simulink model "GFo_29bus"  (R2015b)
settings: Solver=ode1  StartTime=0.0  StopTime=4.5  FixedStep=Time_Step  RelTol=1e-3
PreLoadFcn:
  | Init_29bus;
InitFcn:
  | Init_29bus;
undefined symbols (not defined in the file): C_line, D1, D11, Delta, DX_DR, fb, fn, I_thresh_pu, Kp_Rvi_pu, Time_Step, VSC01_Cf, VSC01_Cf_pu, VSC01_Delta_P_Time_Step, VSC01_Delta_P_Value, VSC01_id0, VSC01_Lf, VSC01_Lf_pu, VSC01_Lt_pu, VSC01_mp1, VSC01_mp2, VSC01_mp3, VSC01_Pn, VSC01_R, VSC01_Rf, VSC01_Rf_pu, VSC01_Rt_pu, VSC01_Rv, VSC01_Sn, VSC01_T1, VSC01_T2, VSC01_Tr_PLL, VSC01_Udc_n, VSC01_Udcb, VSC01_Un1, VSC01_Un2, VSC01_W_LF, VSC01_wc1, VSC01_wc2, VSC01_wc3
libraries: powerlib x183, sps_avr x6, simulink x4, powerlib_meascontrol x2
(part 3 of 6)

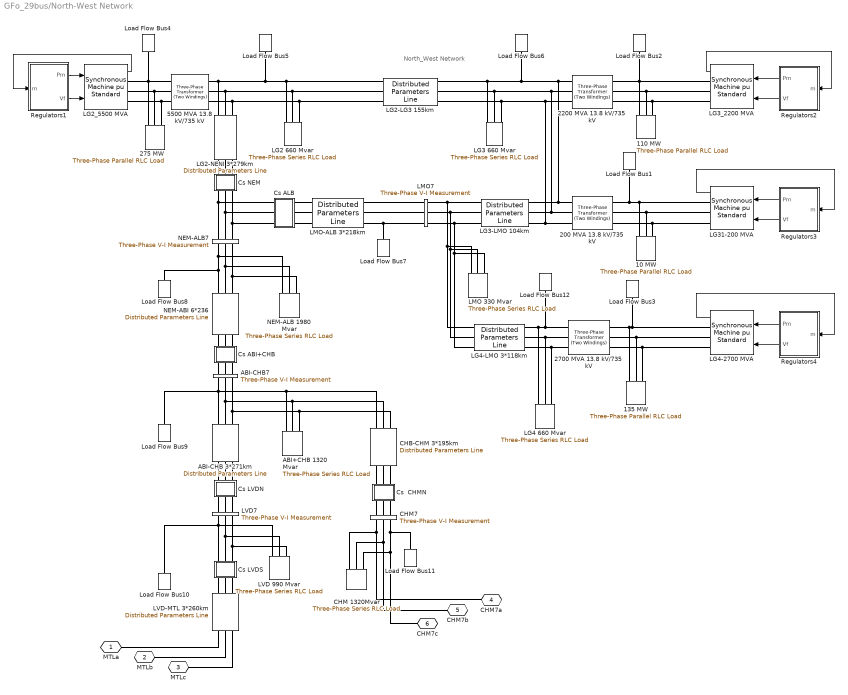
== system GFo_29bus/North-West Network ==
  note: North_West Network
  10 MW : powerlib/Elements/Three-Phase Parallel RLC Load  LConnTagsString=A|B|C  Configuration=Y (grounded)  NominalVoltage=(13800)*1  Vabc=[1e3 1e3 1e3]  Vabcp=[1e3 1e3 1e3]  NominalFrequency=60  UnbalancedPower=off  ActivePower=10000000  InductivePower=0  CapacitivePower=0  Pabc=[10e3 9e3 11e3]  QLabc=[100 90 110]  QCabc=[100 90 110]  Pabcp=[10e3 9e3 11e3]  QLabcp=[100 90 110]  QCabcp=[100 90 110]  Measurements=None  LoadType=constant PQ
  110 MW : powerlib/Elements/Three-Phase Parallel RLC Load  LConnTagsString=A|B|C  Configuration=Y (grounded)  NominalVoltage=(13800)*1  Vabc=[1e3 1e3 1e3]  Vabcp=[1e3 1e3 1e3]  NominalFrequency=60  UnbalancedPower=off  ActivePower=110000000  InductivePower=0  CapacitivePower=0  Pabc=[10e3 9e3 11e3]  QLabc=[100 90 110]  QCabc=[100 90 110]  Pabcp=[10e3 9e3 11e3]  QLabcp=[100 90 110]  QCabcp=[100 90 110]  Measurements=None  LoadType=constant PQ
  135 MW : powerlib/Elements/Three-Phase Parallel RLC Load  LConnTagsString=A|B|C  Configuration=Y (grounded)  NominalVoltage=(13800)*1  Vabc=[1e3 1e3 1e3]  Vabcp=[1e3 1e3 1e3]  NominalFrequency=60  UnbalancedPower=off  ActivePower=135000000  InductivePower=0  CapacitivePower=0  Pabc=[10e3 9e3 11e3]  QLabc=[100 90 110]  QCabc=[100 90 110]  Pabcp=[10e3 9e3 11e3]  QLabcp=[100 90 110]  QCabcp=[100 90 110]  Measurements=None  LoadType=constant PQ
  200 MVA 13.8 kV/735 kV : powerlib/Elements/Three-Phase Transformer (Two Windings)  Winding1Connection=Delta (D1)  Winding2Connection=Yg  CoreType=Three single-phase transformers  SetSaturation=off  Hysteresis=off  DataFile='basic_model'  SetInitialFlux=off  Measurements=None  UNITS=pu  NominalPower=[ 200e6 60 ]  Winding1="[ 13.8e3 0.002  0.0]"  Winding2=[ 735e3 0.002 0.12]  Rm=500  Lm=500  L0=0.5  Saturation="[ 0,0  ;  0.005,1.2  ;  1.0,1.4 ]"  InitialFluxes=[ 0.8 , -0.8 , 0.7 ]  MoreParameters=off  BreakLoop=off  DataType=off  TransfoNumber=0
  2200 MVA 13.8 kV/735 kV : powerlib/Elements/Three-Phase Transformer (Two Windings)  Winding1Connection=Delta (D1)  Winding2Connection=Yg  CoreType=Three single-phase transformers  SetSaturation=off  Hysteresis=off  DataFile='basic_model'  SetInitialFlux=off  Measurements=None  UNITS=pu  NominalPower=[ 2200e6 60 ]  Winding1="[ 13.8e3 0.002  0.0]"  Winding2=[ 735e3 0.002 0.12]  Rm=500  Lm=500  L0=0.5  Saturation="[ 0,0  ;  0.005,1.2  ;  1.0,1.4 ]"  InitialFluxes=[ 0.8 , -0.8 , 0.7 ]  MoreParameters=off  BreakLoop=off  DataType=off  TransfoNumber=0
  2700 MVA 13.8 kV/735 kV : powerlib/Elements/Three-Phase Transformer (Two Windings)  Winding1Connection=Delta (D1)  Winding2Connection=Yg  CoreType=Three single-phase transformers  SetSaturation=off  Hysteresis=off  DataFile='basic_model'  SetInitialFlux=off  Measurements=None  UNITS=pu  NominalPower=[ 2700e6 60 ]  Winding1="[ 13.8e3 0.002  0.0]"  Winding2=[ 735e3 0.002 0.12]  Rm=500  Lm=500  L0=0.5  Saturation="[ 0,0  ;  0.005,1.2  ;  1.0,1.4 ]"  InitialFluxes=[ 0.8 , -0.8 , 0.7 ]  MoreParameters=off  BreakLoop=off  DataType=off  TransfoNumber=0
  275 MW : powerlib/Elements/Three-Phase Parallel RLC Load  LConnTagsString=A|B|C  Configuration=Y (grounded)  NominalVoltage=(13800)*1  Vabc=[1e3 1e3 1e3]  Vabcp=[1e3 1e3 1e3]  NominalFrequency=60  UnbalancedPower=off  ActivePower=275000000  InductivePower=0  CapacitivePower=0  Pabc=[10e3 9e3 11e3]  QLabc=[100 90 110]  QCabc=[100 90 110]  Pabcp=[10e3 9e3 11e3]  QLabcp=[100 90 110]  QCabcp=[100 90 110]  Measurements=None  LoadType=constant PQ
  5500 MVA 13.8 kV/735 kV : powerlib/Elements/Three-Phase Transformer (Two Windings)  Winding1Connection=Delta (D1)  Winding2Connection=Yg  CoreType=Three single-phase transformers  SetSaturation=off  Hysteresis=off  DataFile='basic_model'  SetInitialFlux=off  Measurements=None  UNITS=pu  NominalPower=[ 5500e6 60 ]  Winding1="[ 13.8e3 0.002  0.0]"  Winding2=[ 735e3 0.002 0.12]  Rm=500  Lm=500  L0=0.5  Saturation="[ 0,0  ;  0.005,1.2  ;  1.0,1.4 ]"  InitialFluxes=[ 0.8 , -0.8 , 0.7 ]  MoreParameters=off  BreakLoop=off  DataType=off  TransfoNumber=0
  ABI+CHB 1320 Mvar : powerlib/Elements/Three-Phase Series RLC Load  LConnTagsString=A|B|C  Configuration=Y (grounded)  NominalVoltage=735e3  Vabc=[1e3 1e3 1e3]  Vabcp=[1e3 1e3 1e3]  NominalFrequency=60  UnbalancedPower=off  ActivePower=4400000  InductivePower=1320e6  CapacitivePower=0  Pabc=[10e3 9e3 11e3]  QLabc=[100 90 110]  QCabc=[100 90 110]  Pabcp=[10e3 9e3 11e3]  QLabcp=[100 90 110]  QCabcp=[100 90 110]  Measurements=None  LoadType=constant Z
  ABI-CHB 3*271km : powerlib/Elements/Distributed Parameters Line  Phases=3  Frequency=60  Resistance="[0.01273  0.3864]/3"  Inductance="[0.9337e-3  4.1264e-3]/3"  Capacitance=[12.74e-9 7.751e-9]*3  Length=271  x1=[-0.00156 -3.49602547978954e-08 0 0;-0.00152 -3.60388902575001e-08 0 0;-0.00148 -3.71093307842464e-08 0 0;-0.00144 -3.81713329691896e-08 0 0;-0.0014 -3.92246553221912e-08 0 0;-0.00136 -4.02690583268316e-08 0 0;-0.00132 -4.1304304494874e-08 0 0;-0.00128 -4.23301584202674e-08 0 0;-0.00124 -4.33463868326757e-08 0 0;-0.0012 -4.43527586505217e-08 0 0;-0.00116 -4.53490450335324e-08 0 0;-0.00112 -4.6335019434776e-08 0 0;-0.00108 -4.73104576521763e-08 0 0;-0.00104 -4.82751378794945e-08 0 0;-0.001 -4.9228840756766e-08 0 0;-0.00096 -5.01713494201809e-08 216587.676799688 -655260.200479363;-0.00092 -5.11024495513968e-08 226443.759556855 -651919.748758476;-0.00088 -5.20219294262736e-08 236248.350955866 -648431.056108637;-0.00084 -5.29295799630168e-08 245999.221517189 -644794.915828471;-0.0008 -5.38251947697217e-08 255694.153976947 -641012.15474492;-0.00076 -5.47085701913047e-08 265330.943791102 -637083.633025233;-0.00072 -5.55795053558128e-08 274907.399636756 -633010.243981371;-0.00068 -5.64378022201002e-08 284421.343910432 -628792.913866876;-0.00064 -5.72832656148616e-08 293870.613223249 -624432.601666247;-0.0006 -5.81157032890121e-08 303253.058892851 -619930.298876876;-0.00056 -5.89349259534031e-08 312566.547432004 -615287.029283592;-0.00052 -5.97407473238655e-08 321808.96103373 -610503.848725858;-0.00048 -6.05329841635687e-08 330978.198052879 -605581.844857685;-0.00044 -6.13114563246873e-08 340072.173484025 -600522.136900307;-0.0004 -6.20759867893652e-08 349088.819435579 -595325.87538768;-0.00036 -6.28264017099676e-08 358026.085600006 -589994.241904861;-0.00032 -6.35625304486131e-08 366881.939720054 -584528.448819327;-0.00028 -6.42842056159744e-08 375654.368050865 -578929.73900529;-0.00024 -6.49912631093421e-08 384341.375817886 -573199.38556108;-0.0002 -6.56835421499394e-08 392940.987670464 -567338.691519655;-0.00016 -6.63608853194826e-08 401451.248131026 -561348.989552299;-0.00012 -6.70231385959761e-08 409870.22203973 -555231.641665587;-8e-05 -6.76701513887358e-08 418195.994994513 -548988.038891673;-4e-05 -6.83017765726322e-08 426426.673786403 -542619.600971986]  x2=[-0.00156 -7.66036881931219e-08 0 0;-0.00152 -7.88179038071448e-08 0 0;-0.00148 -8.10141969095385e-08 0 0;-0.00144 -8.31920680821918e-08 0 0;-0.0014 -8.53510220959809e-08 0 0;-0.00136 -8.74905680233813e-08 0 0;-0.00132 -8.96102193500997e-08 0 0;-0.00128 -9.17094940857036e-08 0 0;-0.00124 -9.37879148732213e-08 0 0;-0.0012 -9.58450090976894e-08 0 0;-0.00116 -9.78803089936208e-08 0 0;-0.00112 -9.98933517513709e-08 0 0;-0.00108 -1.01883679622376e-07 0 0;-0.00104 -1.03850840023243e-07 0 0;-0.001 -1.0579438563866e-07 0 0;-0.00096 -1.07713874523115e-07 -50356.5060781829 -677474.330127236;-0.00092 -1.09608870201388e-07 -40135.0993416283 -678156.632405211;-0.00088 -1.11478941767803e-07 -29904.5662295937 -678684.727713151;-0.00084 -1.13323663984215e-07 -19667.2330770844 -679058.495966737;-0.0008 -1.15142617376698e-07 -9425.42776537653 -679277.852174291;-0.00076 -1.16935388330937e-07 818.520807323877 -679342.746456104;-0.00072 -1.18701569186277e-07 11062.2832554513 -679253.164055774;-0.00068 -1.20440758328423e-07 21303.5302357635 -679009.125343568;-0.00064 -1.22152560280763e-07 31539.9329770139 -678610.685811785;-0.0006 -1.23836585794293e-07 41769.1638094941 -678057.936062137;-0.00056 -1.25492451936135e-07 51988.8966943259 -677351.001785151;-0.00052 -1.27119782176607e-07 62196.8077523827 -676490.043731585;-0.00048 -1.28718206474847e-07 72390.5757927189 -675475.257675877;-0.00044 -1.30287361362953e-07 82567.8828403897 -674306.874371624;-0.0004 -1.31826890028635e-07 92726.4146635376 -672985.159499113;-0.00036 -1.33336442396351e-07 102863.86129963 -671510.413604909;-0.00032 -1.34815675206911e-07 112977.917580722 -669882.972033511;-0.00028 -1.3626425209553e-07 123066.283657637 -668103.204851096;-0.00024 -1.37681843668315e-07 133126.665522926 -666171.516761376;-0.0002 -1.39068127577168e-07 143156.775532512 -664088.347013562;-0.00016 -1.40422788593082e-07 153154.332925872 -661854.169302491;-0.00012 -1.41745518677825e-07 163117.064344672 -659469.491660909;-8e-05 -1.43036017053981e-07 173042.704349701 -656934.856343945;-4e-05 -1.4429399027335e-07 182928.995936018 -654250.839705814]  x3=[-0.00156 3.89449950371453e-10 0 0;-0.00152 3.78955368381599e-10 0 0;-0.00148 3.68374615208948e-10 0 0;-0.00144 3.57710096825525e-10 0 0;-0.0014 3.46964238250845e-10 0 0;-0.00136 3.36139483000479e-10 0 0;-0.00132 3.25238292530421e-10 0 0;-0.00128 3.14263145677378e-10 0 0;-0.00124 3.03216538095098e-10 0 0;-0.0012 2.92100981686883e-10 0 0;-0.00116 2.80919004034404e-10 0 0;-0.00112 2.6967314782295e-10 0 0;-0.00108 2.58365970263243e-10 0 0;-0.00104 2.47000042509952e-10 0 0;-0.001 2.35577949077031e-10 0 0;-0.00096 2.24102287250028e-10 85.100387182329 865.220294474964;-0.00092 2.1257566649548e-10 72.0441612628443 866.405402860482;-0.00088 2.01000707867546e-10 58.9715531223708 867.393498128952;-0.00084 1.89380043411998e-10 45.8855353592663 868.18435559603;-0.0008 1.77716315567723e-10 32.7890836211211 868.777795427549;-0.00076 1.66012176565848e-10 19.6851759281215 869.173682680408;-0.00072 1.5427028782665e-10 6.57679199587353 869.37192733326;-0.00068 1.4249331935437e-10 -6.53308744215846 869.37248430698;-0.00064 1.3068394913008e-10 -19.6414813124451 869.175353474919;-0.0006 1.18844862502727e-10 -32.7454088792621 868.780579662926;-0.00056 1.06978751578516e-10 -45.8418904224844 868.188252639162;-0.00052 9.50883146087413e-11 -58.9279479151482 867.398507093685;-0.00048 8.31762553762313e-11 -72.0006057006291 866.411522607821;-0.00044 7.12452825805302e-11 -85.0568911692805 865.227523613331;-0.0004 5.92981092219635e-11 -98.0938354343793 863.846779341375;-0.00036 4.73374519847248e-11 -111.108474007226 862.269603761295;-0.00032 3.53660306191255e-11 -124.097847471241 860.496355509215;-0.00028 2.33865673231472e-11 -137.059002154916 858.527437806497;-0.00024 1.14017861234367e-11 -149.988990803448 856.363298368048;-0.0002 -5.85587744113456e-13 -162.884873248921 854.004429300512;-0.00016 -1.25728284540605e-11 -175.743717078876 851.451366990373;-0.00012 -2.45572102112405e-11 -188.562598303117 848.704691981985;-8e-05 -3.65360078705908e-11 -201.338602018598 845.765028845558;-4e-05 -4.85064975568245e-11 -214.06882307225 842.633046035138]  x4=[-0.00156 -5.54020599902801e-10 0 0;-0.00152 -5.57562391334411e-10 0 0;-0.00148 -5.60977397886446e-10 0 0;-0.00144 -5.64264843015864e-10 0 0;-0.0014 -5.67423979185994e-10 0 0;-0.00136 -5.70454088036512e-10 0 0;-0.00132 -5.73354480546798e-10 0 0;-0.00128 -5.76124497192605e-10 0 0;-0.00124 -5.78763508096037e-10 0 0;-0.0012 -5.81270913168772e-10 0 0;-0.00116 -5.83646142248519e-10 0 0;-0.00112 -5.85888655228669e-10 0 0;-0.00108 -5.87997942181109e-10 0 0;-0.00104 -5.89973523472174e-10 0 0;-0.001 -5.91814949871717e-10 0 0;-0.00096 -5.93521802655255e-10 -873.234445044949 -15818.0204896519;-0.00092 -5.95093693699182e-10 -634.614399883324 -15829.3897607238;-0.00088 -5.96530265569031e-10 -395.850048879845 -15837.1595650709;-0.00084 -5.97831191600748e-10 -156.995684988917 -15841.3281359068;-0.0008 -5.98996175974972e-10 81.8943783669032 -15841.8945253344;-0.00076 -6.00024953784302e-10 320.765819647312 -15838.8586045616;-0.00072 -6.00917291093536e-10 559.564321546497 -15832.2210639306;-0.00068 -6.01672984992866e-10 798.235583344441 -15821.983412761;-0.00064 -6.02291863644015e-10 1036.72533325442 -15808.1479790062;-0.0006 -6.02773786319315e-10 1274.97934076396 -15790.7179087247;-0.00056 -6.03118643433706e-10 1512.94342896636 -15769.6971653641;-0.00052 -6.03326356569654e-10 1750.56348688009 -15745.0905288602;-0.00048 -6.03396878494983e-10 1987.78548175311 -15716.9035945499;-0.00044 -6.03330193173615e-10 2224.55547134952 -15685.142771899;-0.0004 -6.03126315769217e-10 2460.81961621549 -15649.8152830446;-0.00036 -6.02785292641754e-10 2696.52419192193 -15610.9291611532;-0.00032 -6.02307201336942e-10 2931.61560128097 -15568.4932485934;-0.00028 -6.01692150568623e-10 3166.04038653345 -15522.5171949259;-0.00024 -6.00940280194036e-10 3399.74524150481 -15473.0114547087;-0.0002 -6.00051761182022e-10 3632.6770237264 -15419.9872851203;-0.00016 -5.99026795574141e-10 3864.78276651966 -15363.4567433996;-0.00012 -5.97865616438733e-10 4096.00969104029 -15303.4326841042;-8e-05 -5.96568487817921e-10 4326.30521827966 -15239.9287561877;-4e-05 -5.95135704667566e-10 4555.61698102086 -15172.9593998955]  x5=0.00153261764655846  V1=ones(3,3)  V2=ones(3,3)  I1=ones(3,3)  I2=ones(3,3)  nHarmo=1  Measurements=None
      settings: AttributesFormatString=\n
  ABI-CHB7 : powerlib/Measurements/Three-Phase V-I Measurement  VoltageMeasurement=no  SetLabelV=on  LabelV=Vabc_ABI7  Vpu=on  VpuLL=off  CurrentMeasurement=no  SetLabelI=off  LabelI=A1  Ipu=off  Pbase=100e6  Vbase=500e3  OutputType=Magnitude  PhasorSimulation=off  PSBequivalent=0
  CHB-CHM 3*195km : powerlib/Elements/Distributed Parameters Line  Phases=3  Frequency=60  Resistance="[0.01273  0.3864]/3"  Inductance="[0.9337e-3  4.1264e-3]/3"  Capacitance=[12.74e-9 7.751e-9]*3  Length=195  x1=[-0.00112 -4.6335019434776e-08 0 0;-0.00108 -4.73104576521763e-08 0 0;-0.00104 -4.82751378794945e-08 0 0;-0.001 -4.9228840756766e-08 0 0;-0.00096 -5.01713494201809e-08 0 0;-0.00092 -5.11024495513968e-08 0 0;-0.00088 -5.20219294262736e-08 0 0;-0.00084 -5.29295799630168e-08 0 0;-0.0008 -5.38251947697217e-08 0 0;-0.00076 -5.47085701913047e-08 0 0;-0.00072 -5.55795053558128e-08 0 0;-0.00068 -5.64378022201002e-08 284421.343910432 -628792.913866876;-0.00064 -5.72832656148616e-08 293870.613223249 -624432.601666247;-0.0006 -5.81157032890121e-08 303253.058892851 -619930.298876876;-0.00056 -5.89349259534031e-08 312566.547432004 -615287.029283592;-0.00052 -5.97407473238655e-08 321808.96103373 -610503.848725858;-0.00048 -6.05329841635687e-08 330978.198052879 -605581.844857685;-0.00044 -6.13114563246873e-08 340072.173484025 -600522.136900307;-0.0004 -6.20759867893652e-08 349088.819435579 -595325.87538768;-0.00036 -6.28264017099676e-08 358026.085600006 -589994.241904861;-0.00032 -6.35625304486131e-08 366881.939720054 -584528.448819327;-0.00028 -6.42842056159744e-08 375654.368050865 -578929.73900529;-0.00024 -6.49912631093421e-08 384341.375817886 -573199.38556108;-0.0002 -6.56835421499394e-08 392940.987670464 -567338.691519655;-0.00016 -6.63608853194826e-08 401451.248131026 -561348.989552299;-0.00012 -6.70231385959761e-08 409870.22203973 -555231.641665587;-8e-05 -6.76701513887358e-08 418195.994994513 -548988.038891673;-4e-05 -6.83017765726322e-08 426426.673786403 -542619.600971986]  x2=[-0.00112 -3.4035079791735e-08 0 0;-0.00108 -3.46803398916117e-08 0 0;-0.00104 -3.53177139812674e-08 0 0;-0.001 -3.59470571273309e-08 0 0;-0.00096 -3.65682262225978e-08 0 0;-0.00092 -3.71810800185726e-08 0 0;-0.00088 -3.77854791575872e-08 0 0;-0.00084 -3.83812862044894e-08 0 0;-0.0008 -3.89683656778949e-08 0 0;-0.00076 -3.95465840809941e-08 0 0;-0.00072 -4.01158099319085e-08 0 0;-0.00068 -4.06759137935883e-08 200688.40467491 -641039.156089466;-0.00064 -4.12267683032457e-08 210331.860760861 -637940.078467723;-0.0006 -4.17682482013154e-08 219927.4891955 -634695.938773497;-0.00056 -4.23002303599382e-08 229473.108015669 -631307.474696179;-0.00052 -4.28225938109587e-08 238966.546629967 -627775.456743278;-0.00048 -4.3335219773433e-08 248405.646312322 -624100.68806522;-0.00044 -4.38379916806378e-08 257788.260692864 -620284.00427271;-0.0004 -4.43307952065771e-08 267112.256245996 -616326.27324673;-0.00036 -4.4813518291979e-08 276375.512775535 -612228.394941185;-0.00032 -4.52860511697766e-08 285575.92389683 -607991.301178263;-0.00028 -4.57482863900685e-08 294711.397515733 -603615.955436548;-0.00024 -4.62001188445517e-08 303779.856304324 -599103.352631928;-0.0002 -4.66414457904225e-08 312779.238173277 -594454.518891367;-0.00016 -4.70721668737393e-08 321707.496740762 -589670.511319567;-0.00012 -4.7492184152242e-08 330562.601797777 -584752.417758595;-8e-05 -4.79014021176237e-08 339342.539769792 -579701.356540515;-4e-05 -4.82997277172479e-08 348045.31417463 -574518.47623309]  x3=[-0.00112 -2.96726562445571e-10 0 0;-0.00108 -2.98557921265796e-10 0 0;-0.00104 -3.00321390589379e-10 0 0;-0.001 -3.02016569418604e-10 0 0;-0.00096 -3.03643072284422e-10 0 0;-0.00092 -3.0520052933411e-10 0 0;-0.00088 -3.06688586415364e-10 0 0;-0.00084 -3.08106905156837e-10 0 0;-0.0008 -3.09455163045078e-10 0 0;-0.00076 -3.1073305349787e-10 0 0;-0.00072 -3.11940285933945e-10 0 0;-0.00068 -3.13076585839056e-10 1577.00475277505 -3661.5344585744;-0.00064 -3.14141694828406e-10 1632.03842707261 -3637.33809003913;-0.0006 -3.15135370705393e-10 1686.70098990594 -3612.31462218926;-0.00056 -3.16057387516695e-10 1740.98001147967 -3586.46974514558;-0.00052 -3.16907535603638e-10 1794.86314921235 -3559.80933581025;-0.00048 -3.17685621649878e-10 1848.33815054315 -3532.33945653044;-0.00044 -3.1839146872536e-10 1901.3928557179 -3504.06635371982;-0.0004 -3.19024916326544e-10 1954.01520055417 -3474.99645643815;-0.00036 -3.1958582041291e-10 2006.19321918455 -3445.13637492937;-0.00032 -3.20074053439705e-10 2057.91504677755 -3414.49289911852;-0.00028 -3.20489504386948e-10 2109.16892223563 -3383.07299706775;-0.00024 -3.20832078784677e-10 2159.94319086948 -3350.88381339182;-0.0002 -3.21101698734429e-10 2210.22630704829 -3317.93266763352;-0.00016 -3.21298302926952e-10 2260.00683682506 -3284.22705259923;-0.00012 -3.21421846656148e-10 2309.2734605366 -3249.77463265515;-8e-05 -3.21472301829238e-10 2358.01497537754 -3214.58324198447;-4e-05 -3.21449656973151e-10 2406.22029794773 -3178.66088280594]  x4=[-0.00112 7.78404396619644e-11 0 0;-0.00108 7.25066391557828e-11 0 0;-0.00104 6.71563512651278e-11 0 0;-0.001 6.17907925993268e-11 0 0;-0.00096 5.64111832401498e-11 0 0;-0.00092 5.10187464643733e-11 0 0;-0.00088 4.56147084656178e-11 0 0;-0.00084 4.02002980755216e-11 0 0;-0.0008 3.47767464843158e-11 0 0;-0.00076 2.93452869608612e-11 0 0;-0.00072 2.39071545722147e-11 0 0;-0.00068 1.84635859027851e-11 1976.43464506423 -10995.3468033902;-0.00064 1.30158187731443e-11 2142.0090164811 -10964.2940798932;-0.0006 7.56509195855814e-12 2307.09631351953 -10930.7481704745;-0.00056 2.11264490729919e-12 2471.65899675181 -10894.7167031845;-0.00052 -3.34028254119301e-12 2635.65964604292 -10856.2078712683;-0.00048 -8.79245043824072e-12 2799.06096905947 -10815.2304313021;-0.00044 -1.42426190078816e-11 2961.82580974973 -10771.7937012024;-0.0004 -1.96895489287832e-11 3123.91715679255 -10725.9075581071;-0.00036 -2.51320016160539e-11 3285.29815201344 -10677.5824361293;-0.00032 -3.05687395028862e-11 3445.93209876576 -10626.8293239851;-0.00028 -3.59985263219692e-11 3605.78247027527 -10573.6597624945;-0.00024 -4.14201273866046e-11 3764.81291794598 -10518.0858419572;-0.0002 -4.68323098714643e-11 3922.98727962552 -10460.1201994036;-0.00016 -5.22338430929238e-11 4080.26958782808 -10399.7760157209;-0.00012 -5.76234987889094e-11 4236.6240779131 -10337.0670126561;-8e-05 -6.30000513981944e-11 4392.0151962179 -10272.0074496957;-4e-05 -6.83622783390807e-11 4546.40760814221 -10204.6121208232]  x5=0.0011028060556417  V1=ones(3,3)  V2=ones(3,3)  I1=ones(3,3)  I2=ones(3,3)  nHarmo=1  Measurements=None
      settings: AttributesFormatString=\n
  CHM 1320Mvar : powerlib/Elements/Three-Phase Series RLC Load  LConnTagsString=A|B|C  Configuration=Y (grounded)  NominalVoltage=735e3  Vabc=[1e3 1e3 1e3]  Vabcp=[1e3 1e3 1e3]  NominalFrequency=60  UnbalancedPower=off  ActivePower=4400000  InductivePower=1320e6  CapacitivePower=0  Pabc=[10e3 9e3 11e3]  QLabc=[100 90 110]  QCabc=[100 90 110]  Pabcp=[10e3 9e3 11e3]  QLabcp=[100 90 110]  QCabcp=[100 90 110]  Measurements=None  LoadType=constant Z
  CHM7 : powerlib/Measurements/Three-Phase V-I Measurement  VoltageMeasurement=no  SetLabelV=on  LabelV=Vabc_CHM7  Vpu=on  VpuLL=off  CurrentMeasurement=no  SetLabelI=off  LabelI=A1  Ipu=off  Pbase=100e6  Vbase=735e3  OutputType=Magnitude  PhasorSimulation=off  PSBequivalent=0
  "Cs  CHMN " : Subsystem  mask{Xc=25/3}
      mask prompts: Xc "Condensator Reactance at  60Hz  (ohm):"
      mask help: Series Compensation
      mask init:
      | Cs=1/Xc/(2*pi*60);
      mask Display: disp('Cs')
  "Cs ABI+CHB " : Subsystem  mask{Xc=25/6}
      mask prompts: Xc "Condensator Reactance at  60Hz  (ohm):"
      mask help: Series Compensation
      mask init:
      | Cs=1/Xc/(2*pi*60);
      mask Display: disp('Cs')
  Cs ALB : Subsystem  mask{Xc=16/3}
      mask prompts: Xc "Reactance @ 60Hz du condensateur (ohm):"
      mask init:
      | Cs=1/Xc/(2*pi*60);
      mask Display: disp('Cs')
  "Cs LVDN " : Subsystem  mask{Xc=34/3}
      mask prompts: Xc "Condensator Reactance at  60Hz  (ohm):"
      mask help: Series Compensation
      mask init:
      | Cs=1/Xc/(2*pi*60);
      mask Display: disp('Cs')
  "Cs LVDS " : Subsystem  mask{Xc=34/3}
      mask prompts: Xc "Condensator Reactance at  60Hz  (ohm):"
      mask help: Series Compensation
      mask init:
      | Cs=1/Xc/(2*pi*60);
      mask Display: disp('Cs')
  "Cs NEM " : Subsystem  mask{Xc=16/3}
      mask prompts: Xc "Condensator Reactance at  60Hz  (ohm):"
      mask help: Series Compensation
      mask init:
      | Cs=1/Xc/(2*pi*60);
      mask Display: disp('Cs')
  LG2 660 Mvar : powerlib/Elements/Three-Phase Series RLC Load  LConnTagsString=A|B|C  Configuration=Y (grounded)  NominalVoltage=735e3  Vabc=[1e3 1e3 1e3]  Vabcp=[1e3 1e3 1e3]  NominalFrequency=60  UnbalancedPower=off  ActivePower=2200000  InductivePower=660e6  CapacitivePower=0  Pabc=[10e3 9e3 11e3]  QLabc=[100 90 110]  QCabc=[100 90 110]  Pabcp=[10e3 9e3 11e3]  QLabcp=[100 90 110]  QCabcp=[100 90 110]  Measurements=None  LoadType=constant Z
  LG2-LG3 155km : powerlib/Elements/Distributed Parameters Line  Phases=3  Frequency=60  Resistance="[0.01273  0.3864]"  Inductance="[0.9337e-3  4.1264e-3]"  Capacitance=[12.74e-9 7.751e-9]  Length=155  x1=[-0.00088 -4.23262671580693e-09 492217.122941526 -498797.252764154;-0.00084 -4.28940865142763e-09 499682.540946216 -491318.32934528;-0.0008 -4.34521521251128e-09 507034.335450174 -483727.684375262;-0.00076 -4.40003370912715e-09 514270.834718728 -476027.043901306;-0.00072 -4.45385167602183e-09 521390.39323435 -468218.15898265;-0.00068 -4.50665687545377e-09 528391.39207083 -460302.805292382;-0.00064 -4.55843729997599e-09 535272.239261406 -452282.782713673;-0.0006 -4.60918117516648e-09 542031.370160766 -444159.914930496;-0.00056 -4.65887696230562e-09 548667.24780083 -435936.049012936;-0.00052 -4.70751336099998e-09 555178.363240249 -427613.054997182;-0.00048 -4.75507931175191e-09 561563.235907522 -419192.8254603;-0.00044 -4.80156399847441e-09 567820.413937664 -410677.275089874;-0.0004 -4.84695685095058e-09 573948.474502352 -402068.340248621;-0.00036 -4.89124754723722e-09 579946.024133459 -393367.978534086;-0.00032 -4.93442601601193e-09 585811.699039919 -384578.168333494;-0.00028 -4.97648243886329e-09 591544.165417842 -375700.908373883;-0.00024 -5.01740725252341e-09 597142.119753809 -366738.217267614;-0.0002 -5.05719115104257e-09 602604.289121279 -357692.133053355;-0.00016 -5.09582508790535e-09 607929.43147004 -348564.712732645;-0.00012 -5.13330027808767e-09 613116.335908645 -339358.031802154;-8e-05 -5.16960820005444e-09 618163.822979755 -330074.183781729;-4e-05 -5.20474059769733e-09 623070.744928336 -320715.279738352]  x2=[-0.00088 -6.68954234344848e-09 498836.623614221 -488147.5029039;-0.00084 -6.77458910534282e-09 506140.702918543 -480569.9805379;-0.0008 -6.85809538409617e-09 513329.690191792 -472883.180702585;-0.00076 -6.94004219110087e-09 520401.950720259 -465088.851309949;-0.00072 -7.0204108923597e-09 527355.876332888 -457188.764723281;-0.00068 -7.09918321272305e-09 534189.885766961 -449184.717354143;-0.00064 -7.17634124004457e-09 540902.425027669 -441078.529253882;-0.0006 -7.25186742925423e-09 547491.967741469 -432872.043699768;-0.00056 -7.32574460634793e-09 553957.015503175 -424567.126775847;-0.00052 -7.39795597229267e-09 560296.098216677 -416165.666948607;-0.00048 -7.46848510684657e-09 566507.774429232 -407669.574637564;-0.00044 -7.53731597229265e-09 572590.631659237 -399080.78178084;-0.0004 -7.60443291708567e-09 578543.286717413 -390401.241395866;-0.00036 -7.66982067941118e-09 584364.386021336 -381632.927135275;-0.00032 -7.73346439065591e-09 590052.60590322 -372777.832838115;-0.00028 -7.79534957878876e-09 595606.65291092 -363837.972076468;-0.00024 -7.85546217165163e-09 601025.26410204 -354815.377697575;-0.0002 -7.91378850015928e-09 606307.207331125 -345712.101361591;-0.00016 -7.9703153014076e-09 611451.281529833 -336530.213075052;-0.00012 -8.02502972168946e-09 616456.316980053 -327271.800720173;-8e-05 -8.0779193194175e-09 621321.175579884 -317938.969580082;-4e-05 -8.12897206795333e-09 626044.751102434 -308533.841860097]  x3=[-0.00088 1.32376578464899e-12 1822.53525045153 -2130.11317243652;-0.00084 1.08156186492231e-12 1854.44819935546 -2102.38868894714;-0.0008 8.39112007354538e-13 1885.93946273093 -2074.18614040013;-0.00076 5.96471342952486e-13 1917.00187973622 -2045.5119398118;-0.00072 3.53695046110797e-13 1947.62838704559 -2016.37260744811;-0.00068 1.10838322065759e-13 1977.81202045537 -1986.77476934194;-0.00064 -1.3204360565789e-13 2007.54591646762 -1956.72515578643;-0.0006 -3.74895507804306e-13 2036.82331385081 -1926.23059980458;-0.00056 -6.1766216194521e-13 2065.63755517724 -1895.29803559544;-0.00052 -8.60288365036977e-13 2093.98208833693 -1863.93449695736;-0.00048 -1.10271894597335e-12 2121.85046802746 -1832.14711568856;-0.00044 -1.34489877813085e-12 2149.23635721962 -1799.94311996541;-0.0004 -1.58677279190411e-12 2176.13352859837 -1767.32983269884;-0.00036 -1.82828598722824e-12 2202.5358659789 -1734.3146698691;-0.00032 -2.06938344608534e-12 2228.43736569736 -1700.90513883954;-0.00028 -2.31001034499241e-12 2253.83213797609 -1667.10883664938;-0.00024 -2.5501119674677e-12 2278.71440826287 -1632.93344828631;-0.0002 -2.78963371647283e-12 2303.078518544 -1598.38674493891;-0.00016 -3.0285211268276e-12 2326.91892863091 -1563.47658222961;-0.00012 -3.26671987759499e-12 2350.23021741996 -1528.21089842836;-8e-05 -3.5041758044332e-12 2373.00708412508 -1492.59771264754;-4e-05 -3.74083491191221e-12 2395.24434948321 -1456.64512301848]  x4=[-0.00088 -1.27329221211409e-11 1450.99532516357 -1864.39271134758;-0.00084 -1.27177947276358e-11 1478.94347975619 -1842.30101377444;-0.0008 -1.26997754172833e-11 1506.55533535538 -1819.79039283809;-0.00076 -1.26788682875191e-11 1533.82461326329 -1796.86596725961;-0.00072 -1.26550780924442e-11 1560.74511268128 -1773.5329498557;-0.00068 -1.26284102417439e-11 1587.31071211994 -1749.79664635328;-0.00064 -1.25988707994573e-11 1613.51537079105 -1725.66245418308;-0.0006 -1.2566466482599e-11 1639.35312998121 -1701.13586125228;-0.00056 -1.25312046596311e-11 1664.81811440679 -1676.22244469661;-0.00052 -1.24930933487881e-11 1689.90453354993 -1650.92786961213;-0.00048 -1.24521412162535e-11 1714.60668297526 -1625.25788776711;-0.00044 -1.2408357574189e-11 1738.91894562702 -1599.21833629403;-0.0004 -1.23617523786172e-11 1762.83579310634 -1572.81513636235;-0.00036 -1.23123362271578e-11 1786.35178692836 -1546.05429183204;-0.00032 -1.22601203566173e-11 1809.46157975887 -1518.94188788837;-0.00028 -1.22051166404346e-11 1832.15991663028 -1491.48408965819;-0.00024 -1.21473375859802e-11 1854.44163613651 -1463.68714080804;-0.0002 -1.2086796331713e-11 1876.30167160672 -1435.55736212437;-0.00016 -1.2023506644192e-11 1897.73505225734 -1407.10115007627;-0.00012 -1.19574829149465e-11 1918.73690432244 -1378.32497536096;-8e-05 -1.1888740157203e-11 1939.30245216199 -1349.23538143243;-4e-05 -1.18172940024719e-11 1959.42701934774 -1319.83898301347]  x5=0.000876589428843401  V1=ones(3,3)  V2=ones(3,3)  I1=ones(3,3)  I2=ones(3,3)  nHarmo=1  Measurements=None
      settings: AttributesFormatString=\n
  LG2-NENI 3*279km : powerlib/Elements/Distributed Parameters Line  Phases=3  Frequency=60  Resistance="[0.01273  0.3864]/3"  Inductance="[0.9337e-3  4.1264e-3]/3"  Capacitance=[12.74e-9 7.751e-9]*3  Length=279  x1=[-0.0016 -3.05949440922947e-09 0 0;-0.00156 -3.13142523515607e-09 0 0;-0.00152 -3.20264400198844e-09 0 0;-0.00148 -3.2731345151932e-09 0 0;-0.00144 -3.3428807458355e-09 0 0;-0.0014 -3.41186683422398e-09 0 0;-0.00136 -3.48007709351705e-09 0 0;-0.00132 -3.54749601328995e-09 0 0;-0.00128 -3.61410826306174e-09 0 0;-0.00124 -3.67989869578125e-09 0 0;-0.0012 -3.74485235127143e-09 0 0;-0.00116 -3.80895445963116e-09 0 0;-0.00112 -3.8721904445938e-09 0 0;-0.00108 -3.93454592684169e-09 0 0;-0.00104 -3.99600672727588e-09 0 0;-0.001 -4.0565588702404e-09 469156.230502968 -520546.816624002;-0.00096 -4.11618858670009e-09 476952.23216764 -513413.158168939;-0.00092 -4.17488231737167e-09 484639.779007779 -506162.753989194;-0.00088 -4.23262671580693e-09 492217.122941526 -498797.252764154;-0.00084 -4.28940865142763e-09 499682.540946216 -491318.32934528;-0.0008 -4.34521521251128e-09 507034.335450174 -483727.684375262;-0.00076 -4.40003370912715e-09 514270.834718728 -476027.043901306;-0.00072 -4.45385167602183e-09 521390.39323435 -468218.15898265;-0.00068 -4.50665687545377e-09 528391.39207083 -460302.805292382;-0.00064 -4.55843729997599e-09 535272.239261406 -452282.782713673;-0.0006 -4.60918117516648e-09 542031.370160766 -444159.914930496;-0.00056 -4.65887696230562e-09 548667.24780083 -435936.049012936;-0.00052 -4.70751336099998e-09 555178.363240249 -427613.054997182;-0.00048 -4.75507931175191e-09 561563.235907522 -419192.8254603;-0.00044 -4.80156399847441e-09 567820.413937664 -410677.275089874;-0.0004 -4.84695685095058e-09 573948.474502352 -402068.340248621;-0.00036 -4.89124754723722e-09 579946.024133459 -393367.978534086;-0.00032 -4.93442601601193e-09 585811.699039919 -384578.168333494;-0.00028 -4.97648243886329e-09 591544.165417842 -375700.908373883;-0.00024 -5.01740725252341e-09 597142.119753809 -366738.217267614;-0.0002 -5.05719115104257e-09 602604.289121279 -357692.133053355;-0.00016 -5.09582508790535e-09 607929.43147004 -348564.712732645;-0.00012 -5.13330027808767e-09 613116.335908645 -339358.031802154;-8e-05 -5.16960820005444e-09 618163.822979755 -330074.183781729;-4e-05 -5.20474059769733e-09 623070.744928336 -320715.279738352]  x2=[-0.0016 -2.24433015141576e-08 0 0;-0.00156 -2.31214987165789e-08 0 0;-0.00152 -2.37944382895833e-08 0 0;-0.00148 -2.44619672125152e-08 0 0;-0.00144 -2.5123933695054e-08 0 0;-0.0014 -2.57801872117301e-08 0 0;-0.00136 -2.64305785361532e-08 0 0;-0.00132 -2.70749597749447e-08 0 0;-0.00128 -2.77131844013679e-08 0 0;-0.00124 -2.83451072886465e-08 0 0;-0.0012 -2.89705847429655e-08 0 0;-0.00116 -2.95894745361457e-08 0 0;-0.00112 -3.02016359379851e-08 0 0;-0.00108 -3.080692974826e-08 0 0;-0.00104 -3.14052183283778e-08 0 0;-0.001 -3.19963656326748e-08 282230.706828565 -628834.165902495;-0.00096 -3.25802372393518e-08 291680.843809443 -624506.879482045;-0.00092 -3.31567003810406e-08 301064.655081788 -620037.585582718;-0.00088 -3.37256239749939e-08 310380.006847838 -615427.300483406;-0.00084 -3.42868786528928e-08 319624.780876934 -610677.072523183;-0.0008 -3.48403367902634e-08 328796.874987185 -605787.981862923;-0.00076 -3.53858725354982e-08 337894.203523488 -600761.140239681;-0.00072 -3.59233618384731e-08 346914.697831784 -595597.690713891;-0.00068 -3.64526824787559e-08 355856.306729459 -590298.807409449;-0.00064 -3.69737140933976e-08 364716.996971758 -584865.695246722;-0.0006 -3.74863382043021e-08 373494.753714131 -579299.589668563;-0.00056 -3.79904382451674e-08 382187.580970391 -573601.756359381;-0.00052 -3.84858995879914e-08 390793.502066583 -567773.490957332;-0.00048 -3.89726095691373e-08 399310.560090465 -561816.118759711;-0.00044 -3.94504575149526e-08 407736.81833649 -555730.994421579;-0.0004 -3.99193347669353e-08 416070.360746198 -549519.501647736;-0.00036 -4.03791347064417e-08 424309.292343911 -543183.052878072;-0.00032 -4.08297527789307e-08 432451.739667631 -536723.088966395;-0.00028 -4.12710865177385e-08 440495.851195057 -530141.07885279;-0.00024 -4.17030355673789e-08 448439.797764595 -523438.519229596;-0.0002 -4.21255017063629e-08 456281.772991301 -516616.93420107;-0.00016 -4.25383888695337e-08 464019.993677636 -509677.874936822;-0.00012 -4.29416031699111e-08 471652.700218946 -502622.919319088;-8e-05 -4.33350529200402e-08 479178.157003586 -495453.671583936;-4e-05 -4.37186486528409e-08 486594.65280758 -488171.761956477]  x3=[-0.0016 2.26069456197243e-10 0 0;-0.00156 2.22950163037741e-10 0 0;-0.00152 2.19780172933805e-10 0 0;-0.00148 2.16560206713847e-10 0 0;-0.00144 2.13290996570417e-10 0 0;-0.0014 2.09973285893711e-10 0 0;-0.00136 2.06607829102526e-10 0 0;-0.00132 2.03195391472712e-10 0 0;-0.00128 1.9973674896316e-10 0 0;-0.00124 1.9623268803935e-10 0 0;-0.0012 1.92684005494518e-10 0 0;-0.00116 1.89091508268473e-10 0 0;-0.00112 1.85456013264104e-10 0 0;-0.00108 1.81778347161623e-10 0 0;-0.00104 1.78059346230587e-10 0 0;-0.001 1.74299856139736e-10 537.612076096211 -984.785129000849;-0.00096 1.70500731764697e-10 552.400938609404 -976.565865052084;-0.00092 1.66662836993591e-10 567.06418991286 -968.124538447152;-0.00088 1.62787044530592e-10 581.598495709684 -959.463068670928;-0.00084 1.58874235697481e-10 596.000551024074 -950.583425266945;-0.0008 1.54925300233247e-10 610.267080952852 -941.487627389538;-0.00076 1.50941136091758e-10 624.39484141014 -932.177743344707;-0.00072 1.46922649237583e-10 638.380619865043 -922.655890119797;-0.00068 1.42870753439978e-10 652.221236072149 -912.92423290212;-0.00064 1.38786370065106e-10 665.913542794689 -902.984984586604;-0.0006 1.34670427866524e-10 679.454426520191 -892.840405272604;-0.00056 1.30523862773993e-10 692.840808168468 -882.492801749973;-0.00052 1.26347617680657e-10 706.069643791771 -871.944526974518;-0.00048 1.22142642228636e-10 719.137925266962 -861.197979532958;-0.00044 1.17909892593086e-10 732.042680979529 -850.255603097507;-0.0004 1.13650331264771e-10 744.780976499307 -839.119885870204;-0.00036 1.09364926831206e-10 757.349915247748 -827.793360017116;-0.00032 1.05054653756402e-10 769.746639156569 -816.278601092546;-0.00028 1.00720492159287e-10 781.968329317658 -804.578227453374;-0.00024 9.6363427590831e-11 794.012206624067 -792.694899663666;-0.0002 9.19844508099439e-11 805.87553240196 -780.631319889685;-0.00016 8.75845575581828e-11 817.555609033359 -768.390231285438;-0.00012 8.31647483333299e-11 829.049780569564 -755.974417368912;-8e-05 7.87260281618883e-11 840.355433335088 -743.386701389123;-4e-05 7.4269406370547e-11 851.469996521988 -730.629945684131]  x4=[-0.0016 -2.64835400483653e-10 0 0;-0.00156 -2.64959148896003e-10 0 0;-0.00152 -2.65022647882804e-10 0 0;-0.00148 -2.65025883004935e-10 0 0;-0.00144 -2.64968853526756e-10 0 0;-0.0014 -2.64851572416279e-10 0 0;-0.00136 -2.64674066342218e-10 0 0;-0.00132 -2.64436375667922e-10 0 0;-0.00128 -2.64138554442202e-10 0 0;-0.00124 -2.63780670387035e-10 0 0;-0.0012 -2.6336280488217e-10 0 0;-0.00116 -2.62885052946618e-10 0 0;-0.00112 -2.62347523217051e-10 0 0;-0.00108 -2.61750337923093e-10 0 0;-0.00104 -2.6109363285953e-10 0 0;-0.001 -2.60377557355431e-10 5385.90687638109 -13143.2421918734;-0.00096 -2.59602274240189e-10 5583.4816498283 -13060.5335375424;-0.00092 -2.58767959806499e-10 5779.78678769823 -12974.8550305142;-0.00088 -2.5787480377027e-10 5974.7776518954 -12886.2261533424;-0.00084 -2.56923009227481e-10 6168.40990317881 -12794.6670594695;-0.0008 -2.55912792608003e-10 6360.63951124435 -12700.1985686437;-0.00076 -2.54844383626384e-10 6551.42276473684 -12602.8421621853;-0.00072 -2.53718025229612e-10 6740.7162811897 -12502.6199781015;-0.00068 -2.52533973541875e-10 6928.47701688968 -12399.5548060527;-0.00064 -2.51292497806314e-10 7114.66227666466 -12293.6700821702;-0.0006 -2.49993880323806e-10 7299.22972359216 -12184.989883727;-0.00056 -2.48638416388768e-10 7482.13738862639 -12073.5389236632;-0.00052 -2.4722641422201e-10 7663.34368014165 -11959.342544966;-0.00048 -2.45758194900648e-10 7842.80739338991 -11842.426714907;-0.00044 -2.44234092285093e-10 8020.4877198704 -11722.8180191377;-0.0004 -2.42654452943138e-10 8196.34425660913 -11600.5436556442;-0.00036 -2.41019636071146e-10 8370.33701534618 -11475.6314285622;-0.00032 -2.39330013412377e-10 8542.42643162864 -11348.109741855;-0.00028 -2.37585969172452e-10 8712.5733738073 -11218.0075928544;-0.00024 -2.35787899931991e-10 8880.73915193479 -11085.3545656672;-0.0002 -2.33936214556434e-10 9046.88552656337 -10950.1808244478;-0.00016 -2.32031334103067e-10 9210.97471744022 -10812.5171065392;-0.00012 -2.30073691725278e-10 9372.96941209839 -10672.3947154838;-8e-05 -2.28063732574061e-10 9532.83277434129 -10529.8455139049;-4e-05 -2.26001913696795e-10 9690.52845261896 -10384.9019162616]  x5=0.00157786097191812  V1=ones(3,3)  V2=ones(3,3)  I1=ones(3,3)  I2=ones(3,3)  nHarmo=1  Measurements=None
      settings: AttributesFormatString=\n
  LG2_5500 MVA : powerlib/Machines/Synchronous Machine pu Standard  PresetModel=No  MechanicalLoad=Mechanical power Pm  ShowDetailedParameters=on  RotorType=Salient-pole  Units=per unit standard parameters  MeasurementBus=off  NominalParameters="[5500E6  13800   60 ]"  Reactances1=[ 31 32 33 34 35 36 37 ]  Reactances2=[ 1.305, 0.296, 0.252, 0.474, 0.243, 0.18 ]  dAxisTimeConstants=Short-circuit  qAxisTimeConstants=Open-circuit  TimeConstants1=[]  TimeConstants2=[]  TimeConstants3=[]  TimeConstants4=[]  TimeConstants5=[ 1.01, 0.053, 0.1 ]  TimeConstants6=[]  TimeConstants7=[]  TimeConstants8=[]  StatorResistance=2.8544e-3  Mechanical="[ 4.1  0  32]"  PolePairs=32  InitialConditions=[0 -66.6445 0.909805 0.909805 0.909805 0.518623 -119.481 120.519 1.38126]  SetSaturation=off  Saturation=[0.6404,0.7127,0.8441,0.9214,0.9956,1.082,1.19,1.316,1.457;0.7,0.7698,0.8872,0.9466,0.9969,1.046,1.1,1.151,1.201]  LoadFlowParameters=[2 4000000000 0 0 0]  TsPowergui=0  TsBlock=-1  IterativeModel=Trapezoidal non iterative  IterativeDiscreteModel=Trapezoidal non iterative  BusType=swing  Pref=0  Qref=0  Qmin=-Inf  Qmax=Inf  PLF=0  QLF=0
      settings: AttributesFormatString=\n\n
  LG3 660 Mvar : powerlib/Elements/Three-Phase Series RLC Load  LConnTagsString=A|B|C  Configuration=Y (grounded)  NominalVoltage=735e3  Vabc=[1e3 1e3 1e3]  Vabcp=[1e3 1e3 1e3]  NominalFrequency=60  UnbalancedPower=off  ActivePower=2200000  InductivePower=660e6  CapacitivePower=0  Pabc=[10e3 9e3 11e3]  QLabc=[100 90 110]  QCabc=[100 90 110]  Pabcp=[10e3 9e3 11e3]  QLabcp=[100 90 110]  QCabcp=[100 90 110]  Measurements=None  LoadType=constant Z
  LG3-LMO 104km : powerlib/Elements/Distributed Parameters Line  Phases=3  Frequency=60  Resistance="[0.01273  0.3864]"  Inductance="[0.9337e-3  4.1264e-3]"  Capacitance=[12.74e-9 7.751e-9]  Length=104  x1=[-0.0006 -7.25186742925423e-09 0 0;-0.00056 -7.32574460634793e-09 0 0;-0.00052 -7.39795597229267e-09 0 0;-0.00048 -7.46848510684657e-09 0 0;-0.00044 -7.53731597229265e-09 0 0;-0.0004 -7.60443291708567e-09 0 0;-0.00036 -7.66982067941118e-09 584364.386021336 -381632.927135275;-0.00032 -7.73346439065591e-09 590052.60590322 -372777.832838115;-0.00028 -7.79534957878876e-09 595606.65291092 -363837.972076468;-0.00024 -7.85546217165163e-09 601025.26410204 -354815.377697575;-0.0002 -7.91378850015928e-09 606307.207331125 -345712.101361591;-0.00016 -7.9703153014076e-09 611451.281529833 -336530.213075052;-0.00012 -8.02502972168946e-09 616456.316980053 -327271.800720173;-8e-05 -8.0779193194175e-09 621321.175579884 -317938.969580082;-4e-05 -8.12897206795333e-09 626044.751102434 -308533.841860097]  x2=[-0.0006 -1.65324009255006e-08 0 0;-0.00056 -1.67328981605069e-08 0 0;-0.00052 -1.69295904787699e-08 0 0;-0.00048 -1.71224331541526e-08 0 0;-0.00044 -1.73113823358937e-08 0 0;-0.0004 -1.74963950585785e-08 0 0;-0.00036 -1.76774292519095e-08 536176.088706188 -449713.400463236;-0.00032 -1.78544437502723e-08 542896.38007391 -441577.210860367;-0.00028 -1.80273983020965e-08 549493.221486543 -433340.610407747;-0.00024 -1.81962535790084e-08 555965.112879237 -425005.472037292;-0.0002 -1.83609711847742e-08 562310.582599701 -416573.691087585;-0.00016 -1.85215136640309e-08 568528.187742842 -408047.184872905;-0.00012 -1.86778445108032e-08 574616.514478868 -399427.892247233;-8e-05 -1.88299281768045e-08 580574.178374784 -390717.773163383;-4e-05 -1.89777300795208e-08 586399.824709195 -381918.808227323]  x3=[-0.0006 2.80245155121487e-11 0 0;-0.00056 2.69335148461138e-11 0 0;-0.00052 2.58363897310676e-11 0 0;-0.00048 2.47333896438001e-11 0 0;-0.00044 2.36247653970192e-11 0 0;-0.0004 2.25107690823184e-11 0 0;-0.00036 2.13916540128529e-11 149.593209238903 -301.85142136535;-0.00032 2.02676746657386e-11 154.128074649701 -299.561213214149;-0.00028 1.91390866241863e-11 158.627892665468 -297.202887426369;-0.00024 1.80061465193841e-11 163.091640066392 -294.776980264957;-0.0002 1.68691119721418e-11 167.518301834806 -292.284043360281;-0.00016 1.572824153431e-11 171.906871386 -289.724643584696;-0.00012 1.4583794629988e-11 176.256350797102 -287.099362923638;-8e-05 1.34360314965323e-11 180.565751034004 -284.408798343291;-4e-05 1.22852131253818e-11 184.834092176252 -281.653561654837]  x4=[-0.0006 -5.44037564814203e-11 0 0;-0.00056 -5.37356587504465e-11 0 0;-0.00052 -5.30553419940694e-11 0 0;-0.00048 -5.23629609104526e-11 0 0;-0.00044 -5.16586729410838e-11 0 0;-0.0004 -5.09426382349735e-11 0 0;-0.00036 -5.02150196122392e-11 3766.92172817366 -3037.36970585386;-0.00032 -4.9475982527081e-11 3812.29384430628 -2980.222658824;-0.00028 -4.87256950301588e-11 3856.79907769454 -2922.39793486186;-0.00024 -4.79643277303793e-11 3900.42730823214 -2863.90868281103;-0.0002 -4.71920537561006e-11 3943.16861523571 -2804.76820262302;-0.00016 -4.64090487157647e-11 3985.01327970061 -2744.98994233303;-0.00012 -4.56154906579655e-11 4025.95178651099 -2684.58749500193;-8e-05 -4.48115600309619e-11 4065.97482660346 -2623.57459562537;-4e-05 -4.39974396416456e-11 4105.07329908382 -2561.96511801051]  x5=0.000588163229675572  V1=ones(3,3)  V2=ones(3,3)  I1=ones(3,3)  I2=ones(3,3)  nHarmo=1  Measurements=None
      settings: AttributesFormatString=\n
  LG31-200 MVA : powerlib/Machines/Synchronous Machine pu Standard  PresetModel=No  MechanicalLoad=Mechanical power Pm  ShowDetailedParameters=on  RotorType=Salient-pole  Units=per unit standard parameters  MeasurementBus=off  NominalParameters="[200E6  13800   60 ]"  Reactances1=[ 31 32 33 34 35 36 37 ]  Reactances2=[ 1.305, 0.296, 0.252, 0.474, 0.243, 0.18 ]  dAxisTimeConstants=Short-circuit  qAxisTimeConstants=Open-circuit  TimeConstants1=[]  TimeConstants2=[]  TimeConstants3=[]  TimeConstants4=[]  TimeConstants5=[ 1.01, 0.053, 0.1 ]  TimeConstants6=[]  TimeConstants7=[]  TimeConstants8=[]  StatorResistance=2.8544e-3  Mechanical="[ 3.2  0  32]"  PolePairs=32  InitialConditions=[0 -66.4984 0.901558 0.901558 0.901558 -2.40403 -122.404 117.596 1.43997]  SetSaturation=off  Saturation=[0.6404,0.7127,0.8441,0.9214,0.9956,1.082,1.19,1.316,1.457;0.7,0.7698,0.8872,0.9466,0.9969,1.046,1.1,1.151,1.201]  LoadFlowParameters=[1 180000000 0 0 0]  TsPowergui=0  TsBlock=-1  IterativeModel=Trapezoidal non iterative  IterativeDiscreteModel=Trapezoidal non iterative  BusType=PV  Pref=180000000  Qref=0  Qmin=-Inf  Qmax=Inf  PLF=0  QLF=0
      settings: AttributesFormatString=\n\n
  LG3_2200 MVA : powerlib/Machines/Synchronous Machine pu Standard  PresetModel=No  MechanicalLoad=Mechanical power Pm  ShowDetailedParameters=on  RotorType=Salient-pole  Units=per unit standard parameters  MeasurementBus=off  NominalParameters="[2200E6  13800   60 ]"  Reactances1=[ 31 32 33 34 35 36 37 ]  Reactances2=[ 1.305, 0.296, 0.252, 0.474, 0.243, 0.18 ]  dAxisTimeConstants=Short-circuit  qAxisTimeConstants=Open-circuit  TimeConstants1=[]  TimeConstants2=[]  TimeConstants3=[]  TimeConstants4=[]  TimeConstants5=[ 1.01, 0.053, 0.1 ]  TimeConstants6=[]  TimeConstants7=[]  TimeConstants8=[]  StatorResistance=2.8544e-3  Mechanical="[ 3.2  0  32]"  PolePairs=32  InitialConditions=[0 -68.8829 0.819574 0.819574 0.819574 -2.94125 -122.941 117.059 1.37348]  SetSaturation=off  Saturation=[0.6404,0.7127,0.8441,0.9214,0.9956,1.082,1.19,1.316,1.457;0.7,0.7698,0.8872,0.9466,0.9969,1.046,1.1,1.151,1.201]  LoadFlowParameters=[1 1800000000 0 0 0]  TsPowergui=0  TsBlock=-1  IterativeModel=Trapezoidal non iterative  IterativeDiscreteModel=Trapezoidal non iterative  BusType=PV  Pref=1800000000  Qref=0  Qmin=-Inf  Qmax=Inf  PLF=0  QLF=0
      settings: AttributesFormatString=\n\n
  LG4 660 Mvar : powerlib/Elements/Three-Phase Series RLC Load  LConnTagsString=A|B|C  Configuration=Y (grounded)  NominalVoltage=735e3  Vabc=[1e3 1e3 1e3]  Vabcp=[1e3 1e3 1e3]  NominalFrequency=60  UnbalancedPower=off  ActivePower=2200000  InductivePower=660e6  CapacitivePower=0  Pabc=[10e3 9e3 11e3]  QLabc=[100 90 110]  QCabc=[100 90 110]  Pabcp=[10e3 9e3 11e3]  QLabcp=[100 90 110]  QCabcp=[100 90 110]  Measurements=None  LoadType=constant Z
  LG4-2700 MVA : powerlib/Machines/Synchronous Machine pu Standard  PresetModel=No  MechanicalLoad=Mechanical power Pm  ShowDetailedParameters=on  RotorType=Salient-pole  Units=per unit standard parameters  MeasurementBus=off  NominalParameters="[2700E6  13800   60 ]"  Reactances1=[ 31 32 33 34 35 36 37 ]  Reactances2=[ 1.305, 0.296, 0.252, 0.474, 0.243, 0.18 ]  dAxisTimeConstants=Short-circuit  qAxisTimeConstants=Open-circuit  TimeConstants1=[]  TimeConstants2=[]  TimeConstants3=[]  TimeConstants4=[]  TimeConstants5=[ 1.01, 0.053, 0.1 ]  TimeConstants6=[]  TimeConstants7=[]  TimeConstants8=[]  StatorResistance=2.8544e-3  Mechanical="[ 3.7  0  32]"  PolePairs=32  InitialConditions=[0 -68.039 0.926343 0.926343 0.926343 -0.242764 -120.243 119.757 1.37337]  SetSaturation=off  Saturation=[0.6404,0.7127,0.8441,0.9214,0.9956,1.082,1.19,1.316,1.457;0.7,0.7698,0.8872,0.9466,0.9969,1.046,1.1,1.151,1.201]  LoadFlowParameters=[1 2500000000 0 0 0]  TsPowergui=0  TsBlock=-1  IterativeModel=Trapezoidal non iterative  IterativeDiscreteModel=Trapezoidal non iterative  BusType=PV  Pref=2500000000  Qref=0  Qmin=-Inf  Qmax=Inf  PLF=0  QLF=0
      settings: AttributesFormatString=\n\n
  LG4-LMO 3*118km : powerlib/Elements/Distributed Parameters Line  Phases=3  Frequency=60  Resistance="[0.01273  0.3864]/3"  Inductance="[0.9337e-3  4.1264e-3]/3"  Capacitance=[12.74e-9 7.751e-9]*3  Length=118  x1=[-0.00068 -7.77868802192357e-09 0 0;-0.00064 -7.87206511050075e-09 0 0;-0.0006 -7.9636521593576e-09 0 0;-0.00056 -8.05342834238902e-09 0 0;-0.00052 -8.14137324526519e-09 0 0;-0.00048 -8.2274668700736e-09 0 0;-0.00044 -8.3116896398664e-09 549431.43073737 -430460.013778027;-0.0004 -8.39402240311206e-09 555859.891883546 -422126.138623302;-0.00036 -8.47444643805022e-09 562161.95528384 -413696.275624915;-0.00032 -8.55294345694888e-09 568336.18790338 -405172.341661016;-0.00028 -8.62949561026287e-09 574381.185774913 -396556.275000681;-0.00024 -8.70408549069269e-09 580295.574318054 -387850.034863165;-0.0002 -8.77669613714276e-09 586078.008651851 -379055.600972399;-0.00016 -8.84731103857825e-09 591727.173900601 -370174.973106807;-0.00012 -8.91591413777953e-09 597241.785492845 -361210.170644584;-8e-05 -8.98248983499345e-09 602620.589453461 -352163.232104501;-4e-05 -9.04702299148058e-09 607862.362688814 -343036.214682363]  x2=[-0.00068 -1.6120174925465e-08 0 0;-0.00064 -1.63281443650931e-08 0 0;-0.0006 -1.65324009255006e-08 0 0;-0.00056 -1.67328981605069e-08 0 0;-0.00052 -1.69295904787699e-08 0 0;-0.00048 -1.71224331541526e-08 0 0;-0.00044 -1.73113823358937e-08 522371.29637466 -465677.169975575;-0.0004 -1.74963950585785e-08 529333.87551968 -457747.329117004;-0.00036 -1.76774292519095e-08 536176.088706188 -449713.400463236;-0.00032 -1.78544437502723e-08 542896.38007391 -441577.210860367;-0.00028 -1.80273983020965e-08 549493.221486543 -433340.610407747;-0.00024 -1.81962535790084e-08 555965.112879237 -425005.472037292;-0.0002 -1.83609711847742e-08 562310.582599701 -416573.691087585;-0.00016 -1.85215136640309e-08 568528.187742842 -408047.184872905;-0.00012 -1.86778445108032e-08 574616.514478868 -399427.892247233;-8e-05 -1.88299281768045e-08 580574.178374784 -390717.773163383;-4e-05 -1.89777300795208e-08 586399.824709195 -381918.808227323]  x3=[-0.00068 6.11550242031903e-11 0 0;-0.00064 5.8407349672664e-11 0 0;-0.0006 5.56463938145057e-11 0 0;-0.00056 5.2872784446268e-11 0 0;-0.00052 5.00871522628028e-11 0 0;-0.00048 4.72901306928462e-11 0 0;-0.00044 4.44823557549827e-11 3084.02450201779 -3354.39076966815;-0.0004 4.16644659130201e-11 3134.25460446778 -3307.50502101966;-0.00036 3.88371019308078e-11 3183.77200444937 -3259.86717425209;-0.00032 3.60009067265335e-11 3232.56544213283 -3211.488061801;-0.00028 3.31565252265281e-11 3280.6238223112 -3162.37868465934;-0.00024 3.03046042186159e-11 3327.93621692328 -3112.55020987599;-0.0002 2.74457922050401e-11 3374.49186753853 -3062.0139680164;-0.00016 2.45807392549994e-11 3420.28018780348 -3010.78145058617;-0.00012 2.17100968568273e-11 3465.29076584896 -2958.86430741794;-8e-05 1.88345177698499e-11 3509.51336665768 -2906.27434402237;-4e-05 1.59546558759536e-11 3552.93793439158 -2853.02351890361]  x4=[-0.00068 -1.43969317879098e-10 0 0;-0.00064 -1.42598609501938e-10 0 0;-0.0006 -1.41195475430695e-10 0 0;-0.00056 -1.39760234725956e-10 0 0;-0.00052 -1.38293213749082e-10 0 0;-0.00048 -1.36794746087992e-10 0 0;-0.00044 -1.35265172481308e-10 7982.65400111165 -7445.33835150267;-0.0004 -1.3370484074088e-10 8094.01533465097 -7324.12056646019;-0.00036 -1.32114105672689e-10 8203.536158903 -7201.23733956142;-0.00032 -1.30493328996171e-10 8311.19156977678 -7076.71661339246;-0.00028 -1.28842879261965e-10 8416.95708736025 -6950.58670289261;-0.00024 -1.2716313176811e-10 8520.80866148681 -6822.87628891584;-0.0002 -1.25454468474698e-10 8622.72267720407 -6693.61441170895;-0.00016 -1.23717277917029e-10 8722.67596014373 -6562.83046430811;-0.00012 -1.21951955117253e-10 8820.6457817912 -6430.55418585512;-8e-05 -1.20158901494553e-10 8916.6098646539 -6296.81565483501;-4e-05 -1.18338524773859e-10 9010.54638732695 -6161.64528223641]  x5=0.000667339049054976  V1=ones(3,3)  V2=ones(3,3)  I1=ones(3,3)  I2=ones(3,3)  nHarmo=1  Measurements=None
      settings: AttributesFormatString=\n
  LMO 330 Mvar : powerlib/Elements/Three-Phase Series RLC Load  LConnTagsString=A|B|C  Configuration=Y (grounded)  NominalVoltage=735e3  Vabc=[1e3 1e3 1e3]  Vabcp=[1e3 1e3 1e3]  NominalFrequency=60  UnbalancedPower=off  ActivePower=1100000  InductivePower=330e6  CapacitivePower=0  Pabc=[10e3 9e3 11e3]  QLabc=[100 90 110]  QCabc=[100 90 110]  Pabcp=[10e3 9e3 11e3]  QLabcp=[100 90 110]  QCabcp=[100 90 110]  Measurements=None  LoadType=constant Z
  LMO-ALB 3*218km : powerlib/Elements/Distributed Parameters Line  Phases=3  Frequency=60  Resistance="[0.01273  0.3864]/3"  Inductance="[0.9337e-3  4.1264e-3]/3"  Capacitance=[12.74e-9 7.751e-9]*3  Length=218  x1=[-0.00124 -1.28467008535231e-08 360468.536952161 -599825.015586504;-0.0012 -1.31013213370899e-08 369472.343325245 -594321.270044599;-0.00116 -1.33529626931657e-08 378392.13487365 -588682.380971094;-0.00112 -1.3601567700676e-08 387225.883313701 -582909.630600737;-0.00108 -1.38470798289862e-08 395971.579927179 -577004.33160718;-0.00104 -1.40894432507553e-08 404627.236018096 -570967.826804489;-0.001 -1.43286028546315e-08 413190.883364898 -564801.488841799;-0.00096 -1.45645042577831e-08 421660.57466803 -558506.719891188;-0.00092 -1.47970938182654e-08 430034.383992729 -552084.951328829;-0.00088 -1.50263186472181e-08 438310.407206966 -545537.643409517;-0.00084 -1.52521266208919e-08 446486.762414432 -538866.284934609;-0.0008 -1.54744663925009e-08 454561.590382462 -532072.392913493;-0.00076 -1.56932874038983e-08 462533.054964813 -525157.512218624;-0.00072 -1.59085398970732e-08 470399.343519179 -518123.215234243;-0.00068 -1.6120174925465e-08 478158.66731938 -510971.101498822;-0.00064 -1.63281443650931e-08 485809.261962098 -503702.797341347;-0.0006 -1.65324009255006e-08 493349.387768086 -496319.955511504;-0.00056 -1.67328981605069e-08 500777.330177759 -488824.254803859;-0.00052 -1.69295904787699e-08 508091.40014107 -481217.399676113;-0.00048 -1.71224331541526e-08 515289.934501582 -473501.119861522;-0.00044 -1.73113823358937e-08 522371.29637466 -465677.169975575;-0.0004 -1.74963950585785e-08 529333.87551968 -457747.329117004;-0.00036 -1.76774292519095e-08 536176.088706188 -449713.400463236;-0.00032 -1.78544437502723e-08 542896.38007391 -441577.210860367;-0.00028 -1.80273983020965e-08 549493.221486543 -433340.610407747;-0.00024 -1.81962535790084e-08 555965.112879237 -425005.472037292;-0.0002 -1.83609711847742e-08 562310.582599701 -416573.691087585;-0.00016 -1.85215136640309e-08 568528.187742842 -408047.184872904;-0.00012 -1.86778445108032e-08 574616.514478868 -399427.892247233;-8e-05 -1.88299281768045e-08 580574.178374784 -390717.773163383;-4e-05 -1.89777300795208e-08 586399.824709195 -381918.808227323]  x2=[-0.00124 -2.77475367045661e-08 229543.747318113 -648299.081420842;-0.0012 -2.83685335700354e-08 239293.384797621 -644764.050551686;-0.00116 -2.89830796756107e-08 248988.609025004 -641082.405897643;-0.00112 -2.95910352788072e-08 258627.215389881 -637254.984632958;-0.00108 -3.01922621357635e-08 268207.012156285 -633282.65708022;-0.00104 -3.07866235326771e-08 277725.820961043 -629166.326512459;-0.001 -3.13739843168919e-08 287181.47730912 -624906.928947749;-0.00096 -3.19542109276308e-08 296571.831065804 -620505.432936364;-0.00092 -3.25271714263661e-08 305894.746945631 -615962.83934054;-0.00088 -3.30927355268214e-08 315148.104997926 -611280.181106888;-0.00084 -3.36507746245976e-08 324329.801088866 -606458.523031507;-0.0008 -3.4201161826416e-08 333437.74737994 -601498.961517865;-0.00076 -3.47437719789733e-08 342469.872802704 -596402.624327479;-0.00072 -3.52784816974002e-08 351424.123529728 -591170.670323479;-0.00068 -3.58051693933177e-08 360298.463441613 -585804.289207086;-0.00064 -3.63237153024858e-08 369090.874589993 -580304.701247088;-0.0006 -3.68340015120366e-08 377799.357656395 -574673.157002361;-0.00056 -3.73359119872864e-08 386421.93240687 -568910.937037502;-0.00052 -3.78293325981214e-08 394956.638142275 -563019.35163164;-0.00048 -3.83141511449499e-08 403401.534144129 -556999.740480489;-0.00044 -3.87902573842153e-08 411754.700115904 -550853.472391714;-0.0004 -3.92575430534644e-08 420014.236619695 -544581.944973675;-0.00036 -3.97159018959657e-08 428178.265508126 -538186.584317623;-0.00032 -4.01652296848713e-08 436244.930351434 -531668.844673422;-0.00028 -4.06054242469167e-08 444212.396859595 -525030.208118858;-0.00024 -4.10363854856547e-08 452078.853299435 -518272.184222636;-0.0002 -4.14580154042159e-08 459842.510906597 -511396.30970111;-0.00016 -4.18702181275929e-08 467501.604292291 -504404.148068852;-0.00012 -4.22728999244411e-08 475054.391844732 -497297.28928312;-8e-05 -4.26659692283924e-08 482499.156125162 -490077.349382314;-4e-05 -4.30493366588768e-08 489834.204258384 -482745.970118505]  x3=[-0.00124 1.41250512566587e-10 928.47754647539 -2076.06619786212;-0.0012 1.37507005816738e-10 959.677003284131 -2061.82936078197;-0.00116 1.33732231159576e-10 990.658237818227 -2047.12368148564;-0.00112 1.29927046946306e-10 1021.41420521212 -2031.95250391779;-0.00108 1.26092318443004e-10 1051.93791182404 -2016.31927787335;-0.00104 1.22228917633861e-10 1082.22241682634 -2000.22755821313;-0.001 1.18337723022906e-10 1112.26083378375 -1983.68100405539;-0.00096 1.14419619434236e-10 1142.04633221928 -1966.68337794387;-0.00092 1.1047549781082e-10 1171.57213916745 -1949.23854499216;-0.00088 1.06506255011902e-10 1200.83154071439 -1931.35047200484;-0.00084 1.02512793609065e-10 1229.81788352449 -1913.02322657544;-0.0008 9.84960216809934e-11 1258.52457635338 -1894.26097616152;-0.00076 9.44568526069855e-11 1286.94509154666 -1875.06798713704;-0.00072 9.0396204859256e-11 1315.07296652427 -1855.44862382218;-0.00068 8.63150017940851e-11 1342.90180524999 -1835.40734749097;-0.00064 8.22141714418552e-11 1370.42527968589 -1814.94871535682;-0.0006 7.80946462960242e-11 1397.63713123124 -1794.07737953625;-0.00056 7.3957363101085e-11 1424.53117214565 -1772.79808599104;-0.00052 6.98032626395578e-11 1451.10128695615 -1751.11567344903;-0.00048 6.56332895180641e-11 1477.34143384776 -1729.03507230386;-0.00044 6.14483919525313e-11 1503.24564603737 -1706.56130349381;-0.0004 5.72495215525769e-11 1528.8080331305 -1683.6994773601;-0.00036 5.30376331051202e-11 1554.02278246078 -1660.45479248485;-0.00032 4.88136843572726e-11 1578.88416041165 -1636.83253450893;-0.00028 4.45786357985533e-11 1603.38651372015 -1612.83807493012;-0.00024 4.03334504424833e-11 1627.52427076246 -1588.47686988159;-0.0002 3.60790936076035e-11 1651.29194282076 -1563.75445889128;-0.00016 3.18165326979702e-11 1674.68412533141 -1538.67646362227;-0.00012 2.75467369831755e-11 1697.69549911381 -1513.24858659442;-8e-05 2.32706773779437e-11 1720.32083158002 -1487.47660988767;-4e-05 1.8989326221354e-11 1742.55497792454 -1461.36639382728]  x4=[-0.00124 -2.37997187821012e-10 3596.04264521639 -12576.6616385887;-0.0012 -2.38204542243208e-10 3785.27795789352 -12521.0066500227;-0.00116 -2.38357731006685e-10 3973.65253100586 -12462.5044925212;-0.00112 -2.38456719277642e-10 4161.12352979998 -12401.1684689701;-0.00108 -2.38501484546998e-10 4347.64832498742 -12337.0125266522;-0.00104 -2.38492016635517e-10 4533.18450243828 -12270.0512540757;-0.001 -2.3842831769612e-10 4717.68987282581 -12200.2998776564;-0.00096 -2.38310402213398e-10 4901.12248121988 -12127.7742582559;-0.00092 -2.38138297000314e-10 5083.4406166272 -12052.4908875744;-0.00088 -2.37912041192109e-10 5264.60282147602 -11974.4668844015;-0.00084 -2.37631686237404e-10 5444.56790104324 -11893.7199907223;-0.0008 -2.37297295886496e-10 5623.29493282172 -11810.2685676844;-0.00076 -2.36908946176868e-10 5800.74327582571 -11724.1315914216;-0.00072 -2.36466725415896e-10 5976.87257983225 -11635.3286487396;-0.00068 -2.35970734160766e-10 6151.64279455649 -11543.8799326615;-0.00064 -2.35421085195613e-10 6325.01417875876 -11449.806237837;-0.0006 -2.34817903505871e-10 6496.94730928137 -11353.128955813;-0.00056 -2.34161326249855e-10 6667.40309001315 -11253.8700701696;-0.00052 -2.33451502727572e-10 6836.34276077949 -11152.0521515214;-0.00048 -2.32688594346768e-10 7003.72790615613 -11047.6983523853;-0.00044 -2.31872774586231e-10 7169.5204642045 -10940.8324019151;-0.0004 -2.31004228956339e-10 7333.68273512662 -10831.4786005064;-0.00036 -2.30083154956877e-10 7496.17738983775 -10719.6618142706;-0.00032 -2.29109762032131e-10 7656.96747845472 -10605.4074693807;-0.00028 -2.28084271523257e-10 7816.01643869796 -10488.7415462894;-0.00024 -2.27006916617954e-10 7973.2881042055 -10369.6905738216;-0.0002 -2.25877942297436e-10 8128.74671275684 -10248.2816231416;-0.00016 -2.24697605280729e-10 8282.35691440503 -10124.542301598;-0.00012 -2.2346617396629e-10 8434.0837795149 -9998.50074644532;-8e-05 -2.22183928370981e-10 8583.89280670574 -9870.1856184463;-4e-05 -2.20851160066393e-10 8731.74993069667 -9739.6260953545]  x5=0.00123288061605072  V1=ones(3,3)  V2=ones(3,3)  I1=ones(3,3)  I2=ones(3,3)  nHarmo=1  Measurements=None
      settings: AttributesFormatString=\n
  LMO7 : powerlib/Measurements/Three-Phase V-I Measurement  VoltageMeasurement=no  SetLabelV=on  LabelV=Vabc_LMO7  Vpu=on  VpuLL=off  CurrentMeasurement=no  SetLabelI=off  LabelI=A1  Ipu=off  Pbase=100e6  Vbase=735e3  OutputType=Magnitude  PhasorSimulation=off  PSBequivalent=0
  LVD 990 Mvar : powerlib/Elements/Three-Phase Series RLC Load  LConnTagsString=A|B|C  Configuration=Y (grounded)  NominalVoltage=735e3  Vabc=[1e3 1e3 1e3]  Vabcp=[1e3 1e3 1e3]  NominalFrequency=60  UnbalancedPower=off  ActivePower=3300000  InductivePower=990e6  CapacitivePower=0  Pabc=[10e3 9e3 11e3]  QLabc=[100 90 110]  QCabc=[100 90 110]  Pabcp=[10e3 9e3 11e3]  QLabcp=[100 90 110]  QCabcp=[100 90 110]  Measurements=None  LoadType=constant Z
  LVD-MTL 3*260km : powerlib/Elements/Distributed Parameters Line  Phases=3  Frequency=60  Resistance="[0.01273  0.3864]/3"  Inductance="[0.9337e-3  4.1264e-3]/3"  Capacitance=[12.74e-9 7.751e-9]*3  Length=260  x1=[-0.00148 -7.16480292734697e-08 6552.33030400431 -685039.790964518;-0.00144 -7.36819183680431e-08 16881.3419986295 -684863.095646298;-0.0014 -7.56990528297853e-08 27206.5150216625 -684530.668366136;-0.00136 -7.76989739797149e-08 37525.5015177986 -684042.584715129;-0.00132 -7.9681227053009e-08 47835.9550384958 -683398.955679289;-0.00128 -8.16453613024128e-08 58135.5310755369 -682599.92761431;-0.00124 -8.3590930100736e-08 68421.8875941509 -681645.682212282;-0.0012 -8.55174910424118e-08 78692.6855655713 -680536.436460381;-0.00116 -8.7424606044096e-08 88945.5894989107 -679272.442591525;-0.00112 -8.93118414442835e-08 99178.2679722323 -677853.98802702;-0.00108 -9.11787681019191e-08 109388.394162694 -676281.395311201;-0.00104 -9.30249614939805e-08 119573.646375648 -674555.022038091;-0.001 -9.48500018120112e-08 129731.708572576 -672675.260770084;-0.00096 -9.66534740575815e-08 139860.270897733 -670642.538948683;-0.00092 -9.84349681366552e-08 149957.030203391 -668457.318797299;-0.00088 -1.00194078952842e-07 160019.690573556 -666120.097216152;-0.00084 -1.01930406499511e-07 170045.963846035 -663631.405669272;-0.0008 -1.03643555950753e-07 180033.57013275 -660991.810063657;-0.00076 -1.05333137751155e-07 189980.238338159 -658201.910620584;-0.00072 -1.06998767704388e-07 199883.706675691 -655262.341739128;-0.00068 -1.08640067060562e-07 209741.723182048 -652173.771851901;-0.00064 -1.10256662602359e-07 219552.046229289 -648936.903273063;-0.0006 -1.11848186729893e-07 229312.445034553 -645552.472038614;-0.00056 -1.13414277544302e-07 239020.700167323 -642021.247739031;-0.00052 -1.14954578930041e-07 248674.604054102 -638344.033344267;-0.00048 -1.16468740635857e-07 258271.961480398 -634521.665021165;-0.00044 -1.17956418354437e-07 267810.590089895 -630555.011943319;-0.0004 -1.19417273800695e-07 277288.320880706 -626444.976093432;-0.00036 -1.20850974788702e-07 286702.998698581 -622192.492058213;-0.00032 -1.22257195307216e-07 296052.482726974 -617798.52681586;-0.00028 -1.23635615593818e-07 305334.646973842 -613264.079516176;-0.00024 -1.24985922207623e-07 314547.380755082 -608590.181253374;-0.0002 -1.2630780810055e-07 323688.58917448 -603777.894831614;-0.00016 -1.27600972687148e-07 332756.193600071 -598828.314523327;-0.00012 -1.2886512191294e-07 341748.132136805 -593742.565820394;-8e-05 -1.30099968321295e-07 350662.360095401 -588521.80517821;-4e-05 -1.31305231118787e-07 359496.850457294 -583167.219752725]  x2=[-0.00148 -1.12181664529462e-07 -242142.117577613 -615908.534572222;-0.00144 -1.15133505536214e-07 -232827.258863866 -619489.788463123;-0.0014 -1.18059166176675e-07 -223459.45723927 -622930.17571838;-0.00136 -1.20957981180847e-07 -214040.84286113 -626228.9140236;-0.00132 -1.23829291383195e-07 -204573.557441134 -629385.253274139;-0.00128 -1.26672443872541e-07 -195059.753758342 -632398.475745671;-0.00124 -1.29486792140528e-07 -185501.595169669 -635267.89625739;-0.0012 -1.32271696228628e-07 -175901.255117953 -637992.862327818;-0.00116 -1.35026522873668e-07 -166260.91663773 -640572.754323168;-0.00112 -1.37750645651826e-07 -156582.771858837 -643006.985598249;-0.00108 -1.40443445121073e-07 -146869.021507936 -645295.002629861;-0.00104 -1.43104308962033e-07 -137121.874408088 -647436.285142663;-0.001 -1.45732632117214e-07 -127343.546976489 -649430.346227476;-0.00096 -1.48327816928596e-07 -117536.262720471 -651276.732452005;-0.00092 -1.50889273273533e-07 -107702.2517319 -652975.023963946;-0.00088 -1.53416418698941e-07 -97843.7501800699 -654524.834586455;-0.00084 -1.55908678553744e-07 -87962.9998032174 -655925.81190596;-0.0008 -1.58365486119543e-07 -78062.2473987703 -657177.637352301;-0.00076 -1.60786282739484e-07 -68143.7443124447 -658280.026271167;-0.00072 -1.63170517945292e-07 -58209.7459263092 -659232.727988824;-0.00068 -1.65517649582442e-07 -48262.5111459296 -660035.525869117;-0.00064 -1.67827143933441e-07 -38304.3018867134 -660688.237362731;-0.0006 -1.70098475839188e-07 -28337.3825595705 -661190.714048703;-0.00056 -1.72331128818397e-07 -18364.0195560047 -661542.841668165;-0.00052 -1.74524595185033e-07 -8386.48073275649 -661744.540150334;-0.00048 -1.76678376163759e-07 1592.96510388849 -661795.763630715;-0.00044 -1.78791982003355e-07 11572.048714006 -661696.50046153;-0.0004 -1.80864932088081e-07 21548.500940039 -661446.773214367;-0.00036 -1.82896755046962e-07 31520.0532227846 -661046.63867505;-0.00032 -1.84886988860979e-07 41484.4381172447 -660496.187830721;-0.00028 -1.86835180968128e-07 51439.3898082235 -659795.545849157;-0.00024 -1.88740888366322e-07 61382.6446255543 -658944.8720503;-0.0002 -1.90603677714134e-07 71311.9415588386 -657944.359870038;-0.00016 -1.92423125429329e-07 81225.0227715805 -656794.236816212;-0.00012 -1.94198817785189e-07 91119.6341145989 -655494.764416886;-8e-05 -1.95930351004583e-07 100993.525638602 -654046.238160878;-4e-05 -1.9761733135179e-07 110844.452105806 -652448.987430567]  x3=[-0.00148 2.39801337081057e-10 786.025562543728 795.662303865588;-0.00144 2.25371349571384e-10 773.938496016878 807.424646485536;-0.0014 2.10890114560338e-10 761.675442550196 819.003387703807;-0.00136 1.96360924955881e-10 749.239190656286 830.395894614498;-0.00132 1.81787084570433e-10 736.632568231586 841.599576659784;-0.00128 1.67171907369618e-10 723.858441913318 852.611886218982;-0.00124 1.52518716718697e-10 710.919716427648 863.430319187866;-0.0012 1.3783084462686e-10 697.819333929173 874.052415548073;-0.00116 1.23111630989557e-10 684.5602733319 884.47575992649;-0.00112 1.08364422829036e-10 671.145549631868 894.697982144495;-0.00108 9.35925735332594e-11 657.578213221562 904.716757756907;-0.00104 7.8799442093369e-11 643.861349196283 914.52980858055;-0.001 6.39883923398839e-11 629.998076652621 924.134903212291;-0.00096 4.91627921777933e-11 615.991547979199 933.529857536442;-0.00092 3.43260128207232e-11 601.844948139852 942.712535221407;-0.00088 1.94814280243526e-11 587.561493949388 951.680848205469;-0.00084 4.63241331924996e-12 573.144433342114 960.432757171596;-0.0008 -1.02176547566932e-11 558.597044633285 968.966272011162;-0.00076 -2.50653994260581e-11 543.922635773643 977.279452276481;-0.00072 -3.99074444397482e-11 529.124543597214 985.370407622052;-0.00068 -5.47404148447199e-11 514.206133062548 993.237298234401;-0.00064 -6.95609377514171e-11 499.170796487547 1000.87833525045;-0.0006 -8.43656431007377e-11 484.021952778091 1008.29178116426;-0.00056 -9.91511644303554e-11 468.763046650601 1015.47595022218;-0.00052 -1.13914139640225e-10 453.397547848743 1022.42920880611;-0.00048 -1.28651211757094e-10 437.928950354438 1029.14997580501;-0.00044 -1.4335902969785e-10 422.360771593361 1035.63672297442;-0.0004 -1.58034249031529e-10 406.696551635107 1041.88797528398;-0.00036 -1.72673532739807e-10 390.939852388214 1047.90231125282;-0.00032 -1.87273551975813e-10 375.094256790209 1053.67836327281;-0.00028 -2.01830986821078e-10 359.163367992885 1059.21481791952;-0.00024 -2.16342527040457e-10 343.150808542972 1064.51041625092;-0.0002 -2.30804872834845e-10 327.060219558404 1069.5639540936;-0.00016 -2.45214735591527e-10 310.895259900355 1074.37428231666;-0.00012 -2.59568838631977e-10 294.659605341251 1078.94030709292;-8e-05 -2.73863917956948e-10 278.356947728929 1083.26099014774;-4e-05 -2.88096722988678e-10 261.990994147141 1087.33534899504]  x4=[-0.00148 -5.60391710842773e-10 -5817.9977000365 -14636.6251724598;-0.00144 -5.67476669911001e-10 -5596.62974849147 -14722.6912994089;-0.0014 -5.74432589678202e-10 -5373.98917160492 -14805.4096133196;-0.00136 -5.81257888428205e-10 -5150.12659592406 -14884.7613047607;-0.00132 -5.87951014146935e-10 -4925.09292586808 -14960.7283298418;-0.00128 -5.94510444875321e-10 -4698.93933215296 -15033.2934143165;-0.00124 -6.00934689055382e-10 -4471.71724015563 -15102.4400575104;-0.0012 -6.07222285869392e-10 -4243.47831822033 -15168.1525360731;-0.00116 -6.13371805572058e-10 -4014.27446590967 -15230.4159075537;-0.00112 -6.19381849815629e-10 -3784.15780220309 -15289.2160137984;-0.00108 -6.25251051967874e-10 -3553.18065364548 -15344.5394841701;-0.00104 -6.30978077422837e-10 -3321.39554244855 -15396.3737385889;-0.001 -6.36561623904317e-10 -3088.85517454776 -15444.7069903921;-0.00096 -6.42000421761995e-10 -2855.61242761744 -15489.5282490152;-0.00092 -6.4729323426014e-10 -2621.72033904683 -15530.8273224905;-0.00088 -6.52438857858834e-10 -2387.23209387987 -15568.5948197648;-0.00084 -6.57436122487643e-10 -2152.20101272138 -15602.822152835;-0.0008 -6.62283891811686e-10 -1916.68053961238 -15633.5015387006;-0.00076 -6.66981063490025e-10 -1680.72422987743 -15660.6260011338;-0.00072 -6.71526569426325e-10 -1444.38573794655 -15684.1893722659;-0.00068 -6.75919376011737e-10 -1207.71880515471 -15704.1862939895;-0.00064 -6.80158484359924e-10 -970.777247521506 -15720.6122191769;-0.0006 -6.84242930534204e-10 -733.61494351384 -15733.4634127144;-0.00056 -6.88171785766741e-10 -496.285821794446 -15742.7369523516;-0.00052 -6.91944156669735e-10 -258.843848958962 -15748.4307293653;-0.00048 -6.95559185438574e-10 -21.343017264398 -15750.5434490399;-0.00044 -6.99016050046892e-10 216.162667648237 -15749.074630961;-0.0004 -7.02313964433487e-10 453.619199034355 -15744.0246091253;-0.00036 -7.05452178681067e-10 690.972581326459 -15735.3945318642;-0.00032 -7.08429979186776e-10 928.168842412263 -15723.1863615828;-0.00028 -7.11246688824457e-10 1165.15404590749 -15707.4028743137;-0.00024 -7.13901667098631e-10 1401.87430342054 -15688.0476590859;-0.0002 -7.16394310290131e-10 1638.27578680624 -15665.1251171084;-0.00016 -7.18724051593393e-10 1874.3047404059 -15638.6404607696;-0.00012 -7.20890361245335e-10 2109.90749327092 -15608.5997124518;-8e-05 -7.22892746645824e-10 2345.03047136703 -15575.0097031623;-4e-05 -7.24730752469687e-10 2579.62020975664 -15537.8780709795]  x5=0.00147040807418893  V1=ones(3,3)  V2=ones(3,3)  I1=ones(3,3)  I2=ones(3,3)  nHarmo=1  Measurements=None
      settings: AttributesFormatString=\n
  LVD7 : powerlib/Measurements/Three-Phase V-I Measurement  VoltageMeasurement=no  SetLabelV=on  LabelV=Vabc_LVD7  Vpu=on  VpuLL=off  CurrentMeasurement=no  SetLabelI=off  LabelI=A1  Ipu=off  Pbase=100e6  Vbase=735e3  OutputType=Magnitude  PhasorSimulation=off  PSBequivalent=0
  Load Flow Bus1 : powerlib/Measurements/Load Flow Bus  LConnTagsString=a  Phases=single  Connectors=on one side  ID=LG31_13.8  Vbase=13.8e3  Vref=1  Vangle=0  VLF=1  VLFb=1  VLFc=1  angleLF=0.9651  angleLFb=0  angleLFc=0
      settings: AttributesFormatString=%<ID>\n%<Vbase>V\n%<VLF>pu\n%<angleLF>deg.
  Load Flow Bus10 : powerlib/Measurements/Load Flow Bus  LConnTagsString=a  Phases=single  Connectors=on one side  ID=LVD7  Vbase=735e3  Vref=1  Vangle=0  VLF=1.045  VLFb=1  VLFc=1  angleLF=-9.603  angleLFb=0  angleLFc=0
      settings: AttributesFormatString=%<ID>\n%<Vbase>V\n%<VLF>pu\n%<angleLF>deg.
  Load Flow Bus11 : powerlib/Measurements/Load Flow Bus  LConnTagsString=a  Phases=single  Connectors=on one side  ID=CHM7  Vbase=735e3  Vref=1  Vangle=0  VLF=1.045  VLFb=1  VLFc=1  angleLF=-1.822  angleLFb=0  angleLFc=0
      settings: AttributesFormatString=%<ID>\n%<Vbase>V\n%<VLF>pu\n%<angleLF>deg.
  Load Flow Bus12 : powerlib/Measurements/Load Flow Bus  LConnTagsString=a  Phases=single  Connectors=on one side  ID=LG47  Vbase=735e3  Vref=1  Vangle=0  VLF=1.006  VLFb=1  VLFc=1  angleLF=22.04  angleLFb=0  angleLFc=0
      settings: AttributesFormatString=%<ID>\n%<Vbase>V\n%<VLF>pu\n%<angleLF>deg.
  Load Flow Bus2 : powerlib/Measurements/Load Flow Bus  LConnTagsString=a  Phases=single  Connectors=on one side  ID=LG3_13.8  Vbase=13.8e3  Vref=1  Vangle=0  VLF=1  VLFb=1  VLFc=1  angleLF=0.3986  angleLFb=0  angleLFc=0
      settings: AttributesFormatString=%<ID>\n%<Vbase>V\n%<VLF>pu\n%<angleLF>deg.
  Load Flow Bus3 : powerlib/Measurements/Load Flow Bus  LConnTagsString=a  Phases=single  Connectors=on one side  ID=LG4_13.8  Vbase=13.8e3  Vref=1  Vangle=0  VLF=1  VLFb=1  VLFc=1  angleLF=-1.963  angleLFb=0  angleLFc=0
      settings: AttributesFormatString=%<ID>\n%<Vbase>V\n%<VLF>pu\n%<angleLF>deg.
  Load Flow Bus4 : powerlib/Measurements/Load Flow Bus  LConnTagsString=a  Phases=single  Connectors=on one side  ID=LG2_13.8  Vbase=13.8e3  Vref=1  Vangle=0  VLF=1  VLFb=1  VLFc=1  angleLF=0  angleLFb=0  angleLFc=0
      settings: AttributesFormatString=%<ID>\n%<Vbase>V\n%<VLF>pu\n%<angleLF>deg.
  Load Flow Bus5 : powerlib/Measurements/Load Flow Bus  LConnTagsString=a  Phases=single  Connectors=on one side  ID=LG27  Vbase=735e3  Vref=1  Vangle=0  VLF=1.003  VLFb=1  VLFc=1  angleLF=24.11  angleLFb=0  angleLFc=0
      settings: AttributesFormatString=%<ID>\n%<Vbase>V\n%<VLF>pu\n%<angleLF>deg.
  Load Flow Bus6 : powerlib/Measurements/Load Flow Bus  LConnTagsString=a  Phases=single  Connectors=on one side  ID=LG37  Vbase=735e3  Vref=1  Vangle=0  VLF=0.9957  VLFb=1  VLFc=1  angleLF=25.11  angleLFb=0  angleLFc=0
      settings: AttributesFormatString=%<ID>\n%<Vbase>V\n%<VLF>pu\n%<angleLF>deg.
  Load Flow Bus7 : powerlib/Measurements/Load Flow Bus  LConnTagsString=a  Phases=single  Connectors=on one side  ID=LMO7  Vbase=735e3  Vref=1  Vangle=0  VLF=1.019  VLFb=1  VLFc=1  angleLF=18.66  angleLFb=0  angleLFc=0
      settings: AttributesFormatString=%<ID>\n%<Vbase>V\n%<VLF>pu\n%<angleLF>deg.
  Load Flow Bus8 : powerlib/Measurements/Load Flow Bus  LConnTagsString=a  Phases=single  Connectors=on one side  ID=NEM_ALB7  Vbase=735e3  Vref=1  Vangle=0  VLF=1.032  VLFb=1  VLFc=1  angleLF=10.49  angleLFb=0  angleLFc=0
      settings: AttributesFormatString=%<ID>\n%<Vbase>V\n%<VLF>pu\n%<angleLF>deg.
  Load Flow Bus9 : powerlib/Measurements/Load Flow Bus  LConnTagsString=a  Phases=single  Connectors=on one side  ID=ABI_CHB7  Vbase=735e3  Vref=1  Vangle=0  VLF=1.047  VLFb=1  VLFc=1  angleLF=2.124  angleLFb=0  angleLFc=0
      settings: AttributesFormatString=%<ID>\n%<Vbase>V\n%<VLF>pu\n%<angleLF>deg.
  NEM-ABI 6*236 : powerlib/Elements/Distributed Parameters Line  Phases=3  Frequency=60  Resistance="[0.01273  0.3864]/6"  Inductance="[0.9337e-3  4.1264e-3]/6"  Capacitance=[12.74e-9 7.751e-9]*6  Length=236  x1=[-0.00136 -2.53084535123569e-08 0 0;-0.00132 -2.59373940313527e-08 0 0;-0.00128 -2.65604366106204e-08 0 0;-0.00124 -2.71774395756502e-08 0 0;-0.0012 -2.77882626252888e-08 0 0;-0.00116 -2.83927668636421e-08 0 0;-0.00112 -2.89908148316595e-08 0 0;-0.00108 -2.95822705383903e-08 0 0;-0.00104 -3.01669994919072e-08 0 0;-0.001 -3.07448687298889e-08 0 0;-0.00096 -3.13157468498538e-08 0 0;-0.00092 -3.18795040390406e-08 0 0;-0.00088 -3.2436012103926e-08 0 0;-0.00084 -3.29851444993753e-08 352337.70792848 -596391.126407081;-0.0008 -3.35267763574171e-08 361290.662474422 -591010.375725675;-0.00076 -3.40607845156379e-08 370161.462639355 -585495.234381485;-0.00072 -3.45870475451875e-08 378948.091279821 -579846.956470093;-0.00068 -3.51054457783914e-08 387648.550392238 -574066.826361186;-0.00064 -3.56158613359617e-08 396260.861567236 -568156.158406506;-0.0006 -3.61181781538023e-08 404783.066439521 -562116.296640975;-0.00056 -3.66122820094007e-08 413213.227133198 -555948.614477072;-0.00052 -3.7098060547801e-08 421549.426702424 -549654.514392533;-0.00048 -3.75754033071527e-08 429789.769567305 -543235.427611441;-0.00044 -3.80442017438289e-08 437932.381944936 -536692.813778772;-0.0004 -3.85043492571078e-08 445975.412275481 -530028.160628492;-0.00036 -3.8955741213413e-08 453917.031643202 -523242.983645253;-0.00032 -3.93982749701062e-08 461755.434192342 -516338.825719788;-0.00028 -3.98318498988275e-08 469488.837537755 -509317.256798071;-0.00024 -4.02563674083771e-08 477115.483170212 -502179.873524324;-0.0002 -4.06717309671341e-08 484633.636856264 -494928.298877951;-0.00016 -4.10778461250072e-08 492041.589032598 -487564.181804494;-0.00012 -4.14746205349118e-08 499337.655194772 -480089.196840669;-8e-05 -4.18619639737687e-08 506520.176280258 -472505.043733595;-4e-05 -4.22397883630201e-08 513587.519045703 -464813.447054285]  x2=[-0.00136 -4.16860762368432e-08 0 0;-0.00132 -4.27362110536926e-08 0 0;-0.00128 -4.37766280246897e-08 0 0;-0.00124 -4.48070905679876e-08 0 0;-0.0012 -4.58273643652901e-08 0 0;-0.00116 -4.68372174151344e-08 0 0;-0.00112 -4.78364200856455e-08 0 0;-0.00108 -4.88247451667527e-08 0 0;-0.00104 -4.98019679218558e-08 0 0;-0.001 -5.07678661389273e-08 0 0;-0.00096 -5.17222201810422e-08 0 0;-0.00092 -5.26648130363214e-08 0 0;-0.00088 -5.35954303672781e-08 0 0;-0.00084 -5.45138605595566e-08 196147.053186556 -655036.16496388;-0.0008 -5.54198947700514e-08 206002.083640616 -652003.967322943;-0.00076 -5.63133269743963e-08 215810.270997343 -648823.50960248;-0.00072 -5.71939540138126e-08 225569.384959513 -645495.515011149;-0.00068 -5.80615756413059e-08 235277.206388771 -642020.74030622;-0.00064 -5.89159945672e-08 244931.52781024 -638399.975621497;-0.0006 -5.97570165039995e-08 254530.153914485 -634634.044287645;-0.00056 -6.05844502105685e-08 264070.902056704 -630723.802644972;-0.00052 -6.13981075356177e-08 273551.602753046 -626670.139848708;-0.00048 -6.2197803460488e-08 282970.10017393 -622473.977666816;-0.00044 -6.29833561412224e-08 292324.252634265 -618136.27027039;-0.0004 -6.37545869499156e-08 301611.933080448 -613658.004016684;-0.00036 -6.45113205153326e-08 310831.029574039 -609040.197224826;-0.00032 -6.52533847627863e-08 319979.445771998 -604283.899944258;-0.00028 -6.59806109532661e-08 329055.101403373 -599390.193715965;-0.00024 -6.66928337218078e-08 338055.93274234 -594360.191326542;-0.0002 -6.73898911150956e-08 346979.893077471 -589195.036555155;-0.00016 -6.80716246282895e-08 355824.953177143 -583895.903913457;-0.00012 -6.87378792410676e-08 364589.101750967 -578463.998378513;-8e-05 -6.93885034528766e-08 373270.345907135 -572900.555118799;-4e-05 -7.00233493173813e-08 381866.71160559 -567206.839213335]  x3=[-0.00136 2.600804163195e-10 0 0;-0.00132 2.49332923689497e-10 0 0;-0.00128 2.38528734902803e-10 0 0;-0.00124 2.27670306738776e-10 0 0;-0.0012 2.16760108310342e-10 0 0;-0.00116 2.05800620502538e-10 0 0;-0.00112 1.9479433540838e-10 0 0;-0.00108 1.83743755762186e-10 0 0;-0.00104 1.7265139437047e-10 0 0;-0.001 1.61519773540555e-10 0 0;-0.00096 1.50351424507026e-10 0 0;-0.00092 1.39148886856138e-10 0 0;-0.00088 1.27914707948349e-10 0 0;-0.00084 1.16651442339061e-10 1033.74803242997 -3077.68516647373;-0.0008 1.05361651197745e-10 1080.03959514888 -3061.74661195705;-0.00076 9.40479017255467e-11 1126.08556617771 -3045.11184266418;-0.00072 8.27127665715305e-11 1171.87547505975 -3027.78464119822;-0.00068 7.13588232476805e-11 1217.39890956458 -3009.76894761536;-0.00064 5.99886535427961e-11 1262.64551805577 -2991.06885852894;-0.0006 4.86048429354163e-11 1307.60501184475 -2971.68862617798;-0.00056 3.72099800059033e-11 1352.26716753035 -2951.63265746018;-0.00052 2.58066558478222e-11 1396.6218293235 -2930.90551292986;-0.00048 1.43974634787483e-11 1440.65891135661 -2909.51190576096;-0.00044 2.98499725063787e-12 1484.368399977 -2887.45670067525;-0.0004 -8.42814774010587e-12 1527.74035602388 -2864.74491283617;-0.00036 -1.98393762427348e-11 1570.76491708848 -2841.38170670842;-0.00032 -3.12460934422935e-11 1613.43229975662 -2817.3723948836;-0.00028 -4.26457055496584e-11 1655.73280183345 -2792.72243687217;-0.00024 -5.40356203913421e-11 1697.65680454958 -2767.437437862;-0.0002 -6.54132479989322e-11 1739.19477474831 -2741.52314744383;-0.00016 -7.67760011980272e-11 1780.33726705345 -2714.98545830382;-0.00012 -8.81212961965378e-11 1821.07492601704 -2687.83040488363;-8e-05 -9.9446553172219e-11 1861.39848824673 -2660.06416200823;-4e-05 -1.10749196859299e-10 1901.2987845122 -2631.6930434818]  x4=[-0.00136 -5.34607622139929e-10 0 0;-0.00132 -5.38472079115909e-10 0 0;-0.00128 -5.42214092184683e-10 0 0;-0.00124 -5.4583281044475e-10 0 0;-0.0012 -5.49327411030783e-10 0 0;-0.00116 -5.52697099300745e-10 0 0;-0.00112 -5.55941109016584e-10 0 0;-0.00108 -5.59058702518463e-10 0 0;-0.00104 -5.62049170892507e-10 0 0;-0.001 -5.64911834131996e-10 0 0;-0.00096 -5.67646041291996e-10 0 0;-0.00092 -5.70251170637376e-10 0 0;-0.00088 -5.7272662978419e-10 0 0;-0.00084 -5.75071855834376e-10 6755.55153643353 -26295.7857546725;-0.0008 -5.77286315503753e-10 7151.298594548 -26190.9287766974;-0.00076 -5.79369505243289e-10 7545.41950903224 -26080.1162073795;-0.00072 -5.81320951353604e-10 7937.82466018905 -25963.3732445413;-0.00068 -5.83140210092678e-10 8328.42481847102 -25840.7264345259;-0.00064 -5.84826867776765e-10 8717.13116477055 -25712.2036661602;-0.0006 -5.86380540874452e-10 9103.85531061655 -25577.8341644134;-0.00056 -5.87800876093874e-10 9488.50931827321 -25437.6484837515;-0.00052 -5.89087550463051e-10 9871.00572073632 -25291.6785011893;-0.00048 -5.90240271403327e-10 10251.2575416225 -25139.9574090421;-0.00044 -5.91258776795902e-10 10629.1783149467 -24982.5197073779;-0.0004 -5.92142835041431e-10 11004.6821047843 -24819.4011961722;-0.00036 -5.92892245112695e-10 11377.6835248116 -24650.638967168;-0.00032 -5.93506836600305e-10 11748.0977577223 -24476.2713954407;-0.00028 -5.93986469751457e-10 12115.8405745141 -24296.3381306724;-0.00024 -5.94331035501709e-10 12480.8283536419 -24110.8800881359;-0.0002 -5.9454045549978e-10 12842.9781000322 -23919.9394393908;-0.00016 -5.94614682125369e-10 13202.2074639556 -23723.5596026939;-0.00012 -5.94553698499982e-10 13558.4347597527 -23521.7852331266;-8e-05 -5.94357518490768e-10 13911.5789844084 -23314.6622124405;-4e-05 -5.9402618670737e-10 14261.5598359714 -23102.2376386244]  x5=0.00133467809810995  V1=ones(3,3)  V2=ones(3,3)  I1=ones(3,3)  I2=ones(3,3)  nHarmo=1  Measurements=None
      settings: AttributesFormatString=\n
  NEM-ALB 1980 Mvar : powerlib/Elements/Three-Phase Series RLC Load  LConnTagsString=A|B|C  Configuration=Y (grounded)  NominalVoltage=735e3  Vabc=[1e3 1e3 1e3]  Vabcp=[1e3 1e3 1e3]  NominalFrequency=60  UnbalancedPower=off  ActivePower=6600000  InductivePower=1980e6  CapacitivePower=0  Pabc=[10e3 9e3 11e3]  QLabc=[100 90 110]  QCabc=[100 90 110]  Pabcp=[10e3 9e3 11e3]  QLabcp=[100 90 110]  QCabcp=[100 90 110]  Measurements=None  LoadType=constant Z
  NEM-ALB7 : powerlib/Measurements/Three-Phase V-I Measurement  VoltageMeasurement=no  SetLabelV=on  LabelV=Vabc_NEM7  Vpu=on  VpuLL=off  CurrentMeasurement=no  SetLabelI=off  LabelI=A1  Ipu=off  Pbase=100e6  Vbase=735e3  OutputType=Magnitude  PhasorSimulation=off  PSBequivalent=0
  Regulators1 : Subsystem
  Regulators2 : Subsystem
  Regulators3 : Subsystem
  Regulators4 : Subsystem
  MTLa : PMIOPort  Port=1  Side=Right
  MTLb : PMIOPort  Port=2  Side=Right
  MTLc : PMIOPort  Port=3  Side=Right
  CHM7a : PMIOPort  Port=4  Side=Right
  CHM7b : PMIOPort  Port=5  Side=Right
  CHM7c : PMIOPort  Port=6  Side=Right
  wires:
  Regulators2/1(Pm) -> LG3_2200 MVA/1
  Regulators4/2(Vf) -> LG4-2700 MVA/2
  Regulators4/1(Pm) -> LG4-2700 MVA/1
  Regulators3/2(Vf) -> LG31-200 MVA/2
  Regulators3/1(Pm) -> LG31-200 MVA/1
  Regulators2/2(Vf) -> LG3_2200 MVA/2
  LG3_2200 MVA/1 -> Regulators2/1(m)
  Regulators1/1(Pm) -> LG2_5500 MVA/1
  Regulators1/2(Vf) -> LG2_5500 MVA/2
  LG2_5500 MVA/1 -> Regulators1/1(m)
  LG31-200 MVA/1 -> Regulators3/1(m)
  LG4-2700 MVA/1 -> Regulators4/1(m)
  connections:
  LG2-NENI 3*279km/RConn1 -- "Cs NEM "/LConn1
  LG2-NENI 3*279km/RConn2 -- "Cs NEM "/LConn2
  LG2-NENI 3*279km/RConn3 -- "Cs NEM "/LConn3
  CHB-CHM 3*195km/RConn1 -- "Cs  CHMN "/LConn1
  CHB-CHM 3*195km/RConn2 -- "Cs  CHMN "/LConn2
  CHB-CHM 3*195km/RConn3 -- "Cs  CHMN "/LConn3
  Load Flow Bus2/LConn1 -- 2200 MVA 13.8 kV/735 kV/LConn1 -- LG3_2200 MVA/RConn1 -- 110 MW/LConn1
  2200 MVA 13.8 kV/735 kV/LConn2 -- LG3_2200 MVA/RConn2 -- 110 MW/LConn2
  2200 MVA 13.8 kV/735 kV/LConn3 -- LG3_2200 MVA/RConn3 -- 110 MW/LConn3
  Load Flow Bus1/LConn1 -- 200 MVA 13.8 kV/735 kV/LConn1 -- LG31-200 MVA/RConn1 -- 10 MW/LConn1
  200 MVA 13.8 kV/735 kV/LConn2 -- LG31-200 MVA/RConn2 -- 10 MW/LConn2
  200 MVA 13.8 kV/735 kV/LConn3 -- LG31-200 MVA/RConn3 -- 10 MW/LConn3
  Load Flow Bus6/LConn1 -- 2200 MVA 13.8 kV/735 kV/RConn1 -- 200 MVA 13.8 kV/735 kV/RConn1 -- LG3-LMO 104km/LConn1 -- LG3 660 Mvar/LConn1 -- LG2-LG3 155km/RConn1
  2200 MVA 13.8 kV/735 kV/RConn2 -- LG3 660 Mvar/LConn2 -- LG2-LG3 155km/RConn2 -- 200 MVA 13.8 kV/735 kV/RConn2 -- LG3-LMO 104km/LConn2
  LG3-LMO 104km/RConn1 -- LMO7/RConn1 -- LG4-LMO 3*118km/RConn1 -- LMO 330 Mvar/LConn1
  LG3-LMO 104km/RConn2 -- LMO7/RConn2 -- LG4-LMO 3*118km/RConn2 -- LMO 330 Mvar/LConn2
  LG3-LMO 104km/RConn3 -- LMO7/RConn3 -- LG4-LMO 3*118km/RConn3 -- LMO 330 Mvar/LConn3
  LG4-LMO 3*118km/LConn1 -- LG4 660 Mvar/LConn1 -- 2700 MVA 13.8 kV/735 kV/RConn1 -- Load Flow Bus12/LConn1
  LG4-LMO 3*118km/LConn2 -- 2700 MVA 13.8 kV/735 kV/RConn2 -- LG4 660 Mvar/LConn2
  LG4 660 Mvar/LConn3 -- 2700 MVA 13.8 kV/735 kV/RConn3 -- LG4-LMO 3*118km/LConn3
  Load Flow Bus3/LConn1 -- LG4-2700 MVA/RConn1 -- 2700 MVA 13.8 kV/735 kV/LConn1 -- 135 MW/LConn1
  LG4-2700 MVA/RConn2 -- 2700 MVA 13.8 kV/735 kV/LConn2 -- 135 MW/LConn2
  LG4-2700 MVA/RConn3 -- 2700 MVA 13.8 kV/735 kV/LConn3 -- 135 MW/LConn3
  Load Flow Bus4/LConn1 -- 5500 MVA 13.8 kV/735 kV/LConn1 -- LG2_5500 MVA/RConn1 -- 275 MW/LConn1
  5500 MVA 13.8 kV/735 kV/LConn2 -- LG2_5500 MVA/RConn2 -- 275 MW/LConn2
  LG2_5500 MVA/RConn3 -- 5500 MVA 13.8 kV/735 kV/LConn3 -- 275 MW/LConn3
  5500 MVA 13.8 kV/735 kV/RConn1 -- LG2-NENI 3*279km/LConn1 -- LG2-LG3 155km/LConn1 -- LG2 660 Mvar/LConn1 -- Load Flow Bus5/LConn1
  LG2-LG3 155km/LConn2 -- 5500 MVA 13.8 kV/735 kV/RConn2 -- LG2-NENI 3*279km/LConn2 -- LG2 660 Mvar/LConn2
  LG2-LG3 155km/LConn3 -- 5500 MVA 13.8 kV/735 kV/RConn3 -- LG2-NENI 3*279km/LConn3 -- LG2 660 Mvar/LConn3
  "Cs NEM "/RConn1 -- NEM-ALB7/LConn1 -- Cs ALB/RConn1
  "Cs NEM "/RConn2 -- NEM-ALB7/LConn2 -- Cs ALB/RConn2
  "Cs NEM "/RConn3 -- NEM-ALB7/LConn3 -- Cs ALB/RConn3
  LMO7/LConn1 -- LMO-ALB 3*218km/LConn1
  LMO7/LConn2 -- LMO-ALB 3*218km/LConn2
  Load Flow Bus7/LConn1 -- LMO7/LConn3 -- LMO-ALB 3*218km/LConn3
  Cs ALB/LConn1 -- LMO-ALB 3*218km/RConn1
  Cs ALB/LConn2 -- LMO-ALB 3*218km/RConn2
  Cs ALB/LConn3 -- LMO-ALB 3*218km/RConn3
  200 MVA 13.8 kV/735 kV/RConn3 -- LG3-LMO 104km/LConn3 -- LG3 660 Mvar/LConn3 -- LG2-LG3 155km/RConn3 -- 2200 MVA 13.8 kV/735 kV/RConn3
  Load Flow Bus8/LConn1 -- NEM-ABI 6*236/LConn1 -- NEM-ALB7/RConn1 -- NEM-ALB 1980 Mvar/LConn1
  NEM-ALB 1980 Mvar/LConn2 -- NEM-ALB7/RConn2 -- NEM-ABI 6*236/LConn2
  NEM-ALB 1980 Mvar/LConn3 -- NEM-ALB7/RConn3 -- NEM-ABI 6*236/LConn3
  NEM-ABI 6*236/RConn1 -- "Cs ABI+CHB "/LConn1
  NEM-ABI 6*236/RConn2 -- "Cs ABI+CHB "/LConn2
  NEM-ABI 6*236/RConn3 -- "Cs ABI+CHB "/LConn3
  "Cs ABI+CHB "/RConn1 -- ABI-CHB7/LConn1
  "Cs ABI+CHB "/RConn2 -- ABI-CHB7/LConn2
  "Cs ABI+CHB "/RConn3 -- ABI-CHB7/LConn3
  Load Flow Bus9/LConn1 -- ABI+CHB 1320 Mvar/LConn1 -- CHB-CHM 3*195km/LConn1 -- ABI-CHB 3*271km/LConn1 -- ABI-CHB7/RConn1
  ABI-CHB 3*271km/LConn2 -- ABI-CHB7/RConn2 -- ABI+CHB 1320 Mvar/LConn2 -- CHB-CHM 3*195km/LConn2
  ABI-CHB 3*271km/LConn3 -- ABI-CHB7/RConn3 -- ABI+CHB 1320 Mvar/LConn3 -- CHB-CHM 3*195km/LConn3
  ABI-CHB 3*271km/RConn1 -- "Cs LVDN "/LConn1
  ABI-CHB 3*271km/RConn2 -- "Cs LVDN "/LConn2
  ABI-CHB 3*271km/RConn3 -- "Cs LVDN "/LConn3
  "Cs LVDN "/RConn1 -- LVD7/LConn1
  "Cs LVDN "/RConn2 -- LVD7/LConn2
  "Cs LVDN "/RConn3 -- LVD7/LConn3
  "Cs LVDS "/LConn1 -- LVD 990 Mvar/LConn1 -- Load Flow Bus10/LConn1 -- LVD7/RConn1
  "Cs LVDS "/LConn2 -- LVD7/RConn2 -- LVD 990 Mvar/LConn2
  "Cs LVDS "/LConn3 -- LVD7/RConn3 -- LVD 990 Mvar/LConn3
  "Cs LVDS "/RConn1 -- LVD-MTL 3*260km/LConn1
  "Cs LVDS "/RConn2 -- LVD-MTL 3*260km/LConn2
  "Cs LVDS "/RConn3 -- LVD-MTL 3*260km/LConn3
  MTLa/RConn1 -- LVD-MTL 3*260km/RConn1
  MTLb/RConn1 -- LVD-MTL 3*260km/RConn2
  MTLc/RConn1 -- LVD-MTL 3*260km/RConn3
  "Cs  CHMN "/RConn1 -- CHM7/LConn1
  "Cs  CHMN "/RConn2 -- CHM7/LConn2
  "Cs  CHMN "/RConn3 -- CHM7/LConn3
  CHM 1320Mvar/LConn2 -- CHM7/RConn2 -- CHM7b/RConn1
  Load Flow Bus11/LConn1 -- CHM 1320Mvar/LConn3 -- CHM7c/RConn1 -- CHM7/RConn3
  CHM7a/RConn1 -- CHM 1320Mvar/LConn1 -- CHM7/RConn1
